simulink model "fullCarModel"  (R2024b)
settings: Solver=ode45  StartTime=0.0  StopTime=10.0  RelTol=1e-3  EnableMultiTasking=on
undefined symbols (not defined in the file or in its folder): sigbuilder_block
(part 1 of 2)
settings Model: Creator=Muhammad  LastModifiedBy=ryuu1
settings SolverCC: AlgebraicLoopSolver=TrustRegion
settings DataIOCC: LimitDataPoints=on  SaveFormat=Array  ReturnWorkspaceOutputs=off
settings OptimizationCC: LifeSpan=inf
settings DebuggingCC: UnderspecifiedInitializationDetection=Classic  MergeDetectMultiDrivingBlocksExec=none  SolverPrmCheckMsg=warning  UnconnectedInputMsg=warning  UnconnectedOutputMsg=warning  UnconnectedLineMsg=warning  StateNameClashWarn=warning  SFUnexpectedBacktrackingDiag=warning  SFNoUnconditionalDefaultTransitionDiag=warning  SFExecutionAtInitializationDiag=none  ArithmeticOperatorsInVariantConditions=warning
settings HardwareCC: ProdBitPerPointer=32  ProdBitPerSizeT=32  ProdBitPerPtrDiffT=32  ProdLargestAtomicFloat=None  ProdIntDivRoundTo=Undefined  ProdEndianess=Unspecified  ProdWordSize=32  ProdHWDeviceType=32-bit Generic
settings ModelReferenceCC: PropagateSignalLabelsOutOfModel=off
settings SFSimCC: SimUseLocalCustomCode=off  CustomCodeUndefinedFunction=UseInterfaceOnly
settings RTWCC: RTWUseLocalCustomCode=off  GPUComputeCapability=3.5
settings CodeAppCC: StateflowObjectComments=on
settings GRTTargetCC: TargetLangStandard=C89/C90 (ANSI)
settings ConfigComp: CovMetricSettings=dw  CovSaveCumulativeToWorkspaceVar=on  CovSaveSingleToWorkspaceVar=on  CovExternalEMLEnable=off

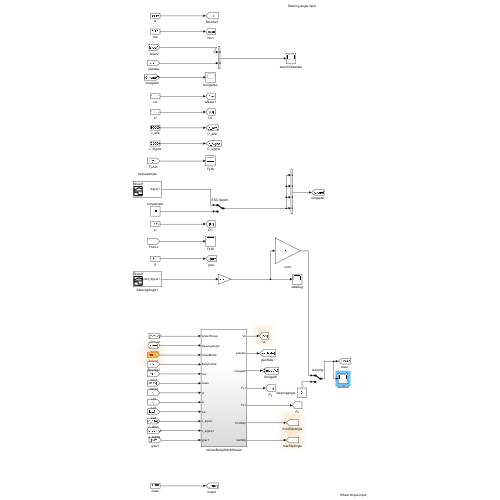
[thumbnail: Simulink's stored preview of the top-level diagram]
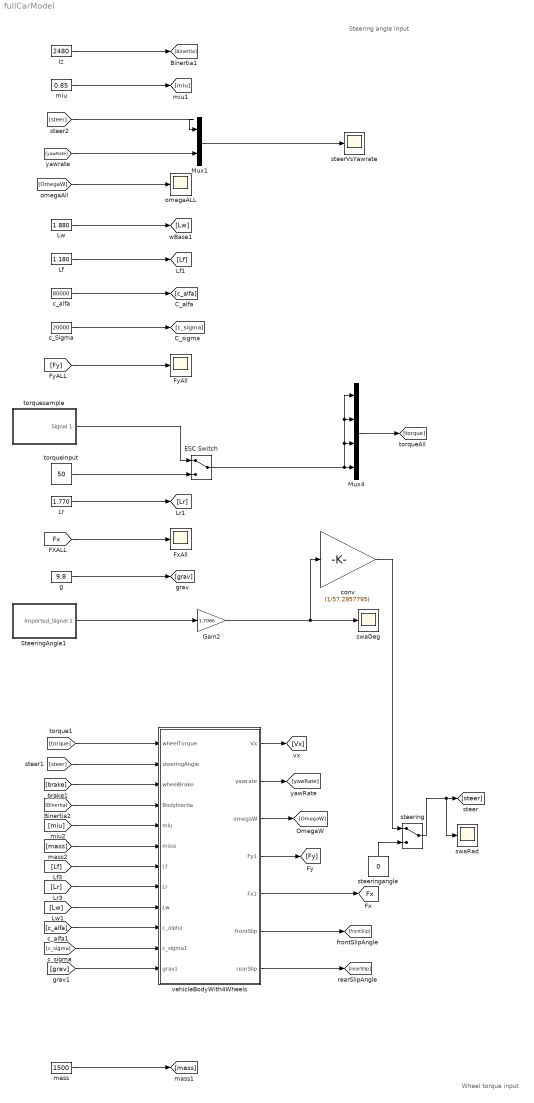
== system fullCarModel ==
  note: Wheel torque input
  note: Steering angle input
  ESC Switch : ManualSwitch
  FxAll : Scope
  FyAll : Scope
  Gain2 : Gain  Gain=1.7086
  Iz : Constant  Value=2480
  Lf : Constant  Value=1.180
  Lr : Constant  Value=1.770
  Lw : Constant  Value=1.880
  Mux1 : Mux  Inputs=2
      settings: DisplayOption=signals
  Mux4 : Mux
      settings: DisplayOption=signals
  SteeringAngle1 : Subsystem  Tag=STV Subsys  LoadFcn=sigbuilder_block('load');  StartFcn=sigbuilder_block('start');  StopFcn=sigbuilder_block('stop');  ClipboardFcn=sigbuilder_block('clipboard');  mask(Sigbuilder block){tuvar=[0:10]}
      mask help: Create and generate interchangeable groups of signals whose waveforms are piecewise linear.
      mask init:
      | if ~strcmp(get_param(bdroot(gcbh),'SimulationStatus'),'stopped') tuvar = sigbuilder_block('maskInit'); end
      settings: CopyFcn=sigbuilder_block('copy');  DeleteFcn=sigbuilder_block('delete');  ModelCloseFcn=sigbuilder_block('modelClose');  PreSaveFcn=sigbuilder_block('preSave');  PauseFcn=sigbuilder_block('pause')  ContinueFcn=sigbuilder_block('continue')  NameChangeFcn=sigbuilder_block('namechange');  OpenFcn=sigbuilder_block('open',[339.75 9 678.75 504 ]);  CloseFcn=sigbuilder_block('close');
      mask Display: plot(0, 0, 100, 100,[2, 2, 32, 32, 2], [68, 8, 8, 68, 68],[32, 2], [38, 38], [32, 19, 2],[53, 60, 44], [32, 17, 17, 2],[16, 16, 31, 31]);txt = getActiveGroup(gcbh);text(2, 100, txt,'verticalAlignment', 'top');
  c_Sigma : Constant  Value=20000
  c_alfa : Constant  Value=80000
  conv : Gain  Gain=(1/57.2957795)
  g : Constant  Value=9.8
  mass : Constant  Value=1500
  miu : Constant  Value=0.85
  omegaALL : Scope
  steerVsYawrate : Scope
  steering : ManualSwitch
  steeringangle : Constant  Value=0
  swaDeg : Scope
  swaRad : Scope
  torqueInput : Constant  Value=50
  "torquesample " : Subsystem  Tag=STV Subsys  LoadFcn=sigbuilder_block('load');  StartFcn=sigbuilder_block('start');  StopFcn=sigbuilder_block('stop');  ClipboardFcn=sigbuilder_block('clipboard');  mask(Sigbuilder block){tuvar=[0:10]}
      mask help: Create and generate interchangeable groups of signals whose waveforms are piecewise linear.
      mask init:
      | if ~strcmp(get_param(bdroot(gcbh),'SimulationStatus'),'stopped') tuvar = sigbuilder_block('maskInit'); end
      settings: CopyFcn=sigbuilder_block('copy');  DeleteFcn=sigbuilder_block('delete');  ModelCloseFcn=sigbuilder_block('modelClose');  PreSaveFcn=sigbuilder_block('preSave');  PauseFcn=sigbuilder_block('pause')  ContinueFcn=sigbuilder_block('continue')  NameChangeFcn=sigbuilder_block('namechange');  OpenFcn=sigbuilder_block('open',[6 28.5 1012.5 484.5 ]);  CloseFcn=sigbuilder_block('close');
      mask Display: plot(0, 0, 100, 100,[2, 2, 32, 32, 2], [68, 8, 8, 68, 68],[32, 2], [38, 38], [32, 19, 2],[53, 60, 44], [32, 17, 17, 2],[16, 16, 31, 31]);txt = getActiveGroup(gcbh);text(2, 100, txt,'verticalAlignment', 'top');
  vehicleBodyWith4Wheels : Subsystem
  tag scope: Fx=global
  wires:
  [steer] -> Mux1/1
  [Fy] -> FyAll/1
  Iz/1 -> [Binertia]
  miu/1 -> [miu]
  Lw/1 -> [Lw]
  Lf/1 -> [Lf]
  vehicleBodyWith4Wheels/5(Fx1) -> [Fx]
  vehicleBodyWith4Wheels/1(Vx) -> [Vx]
  [yawRate] -> Mux1/2
  ESC Switch/1 -> Mux4/2, Mux4/1, Mux4/3, Mux4/4
  [OmegaW] -> omegaALL/1
  Gain2/1 -> swaDeg/1, conv/1
  [c_sigma] -> vehicleBodyWith4Wheels/11(c_sigma1)
  c_alfa/1 -> [c_alfa]
  [mass] -> vehicleBodyWith4Wheels/6(mass)
  c_Sigma/1 -> [c_sigma]
  "torquesample "/1(Signal 1) -> ESC Switch/1
  steering/1 -> swaRad/1, [steer]
  [torque] -> vehicleBodyWith4Wheels/1(wheelTorque)
  torqueInput/1 -> ESC Switch/2
  [Lr] -> vehicleBodyWith4Wheels/8(Lr)
  Lr/1 -> [Lr]
  [Fx] -> FxAll/1
  [grav] -> vehicleBodyWith4Wheels/12(grav1)
  g/1 -> [grav]
  Mux4/1 -> [torque]
  Mux1/1 -> steerVsYawrate/1
  SteeringAngle1/1(Imported_Signal 1) -> Gain2/1
  conv/1 -> steering/1
  [steer] -> vehicleBodyWith4Wheels/2(steeringAngle)
  [brake] -> vehicleBodyWith4Wheels/3(wheelBrake)
  [Binertia] -> vehicleBodyWith4Wheels/4(BodyInertia)
  [miu] -> vehicleBodyWith4Wheels/5(miu)
  [Lf] -> vehicleBodyWith4Wheels/7(Lf)
  [Lw] -> vehicleBodyWith4Wheels/9(Lw)
  [c_alfa] -> vehicleBodyWith4Wheels/10(c_alpha)
  mass/1 -> [mass]
  vehicleBodyWith4Wheels/6(frontSlip) -> [frontSlip]
  vehicleBodyWith4Wheels/2(yawrate) -> [yawRate]
  vehicleBodyWith4Wheels/7(rearSlip) -> [rearSlip]
  vehicleBodyWith4Wheels/3(omegaW) -> [OmegaW]
  vehicleBodyWith4Wheels/4(Fy1) -> [Fy]
  steeringangle/1 -> steering/2

== system fullCarModel/SteeringAngle1 ==
  Demux : Demux  Tag=STV Demux  Outputs=1
      settings: DisplayOption=none
  FromWs : FromWorkspace  Tag=STV FromWs  VariableName=tuvar
      SigBuilderData=|
      | common.afterFinalStr = 'Extrapolate'
      | common.sampleTime = 0
      | dataSet.timeRange = [0 22.075001]
      | dataSet.name = 'Sheet1'
      | sbobj.Name = 'Signal Builder'
      | sbobj.Groups.Name = 'Sheet1'
      | sbobj.Groups.Signals.Name = 'Imported_Signal 1'
      | sbobj.Groups.Signals.XData = [0 8.825 8.85 8.875 8.900001 8.925 8.95 8.975 9 9.025001 9.05 9.075 9.1 9.125 9.150001 9.175 9.2 9.225 9.25 9.275001 9.3 9.325 9.35 9.375 9.400001 9.425 9.45 9.475 9.5 9.525001 9.55 9.575 9.6 9.625 9.650001 9.675 9.7 9.725 9.75 9.775001 9.8 9.825 9.85 9.875 9.900001 9.925 9.95 9.975 10 10.025001 10.05 10.075 10.1 10.125 10.150001 10.175 10.2 10.225 10.25 10.275001 10.3 10.325 10.35 10.375 10.400001 10.425 10.45 10.475 10.5 10.525001 10.55 10.575 10.6 10.625 10.650001 10.675 10.7 10.725 10.75 10.775001 10.8 10.825 10.85 10.875 10.900001 10.925 10.95 10.975 11 11.025001 11.05 11.075 11.1 11.125 11.150001 11.175 11.2 11.225 11.25 11.275001 11.3 11.325 11.35 11.375 11.400001 11.425 11.45 11.475 11.5 11.525001 11.55 11.575 11.6 11.625 11.650001 11.675 11.7 11.725 11.75 11.775001 11.8 11.825 11.85 11.875 11.900001 11.925 11.95 11.975 12 12.025001 12.05 12.075 12.1 12.125 12.150001 12.175 12.2 12.225 12.25 12.275001 12.3 12.325 12.35 12.375 12.400001 12.425 12.45 12.475 12.5 12.525001 12.55 12.575 12.6 12.625 12.650001 12.675 12.7 12.725 12.75 12.775001 12.8 12.825 12.85 12.875 12.900001 12.925 12.95 12.975 13 13.025001 13.05 13.075 13.1 13.125 13.150001 13.175 13.2 13.225 13.25 13.275001 13.3 13.325 13.35 13.375 13.400001 13.425 13.45 13.475 13.5 13.525001 13.55 13.575 13.6 13.625 13.650001 13.675 13.7 13.725 13.75 13.775001 13.8 13.825 13.85 13.875 13.900001 13.925 13.95 13.975 21.85 21.875 21.9 21.925001 21.950001 21.975 22 22.025 22.050001 22.075001]
      | sbobj.Groups.Signals.YData = [0 0.062882 0.050573 0.039906 2.188617 9.974806 17.646795 25.09313 32.23859 39.002769 45.307468 51.033176 56.152084 60.606716 64.344048 67.25927 69.377258 70.674423 71.133003 70.682831 69.396751 67.289543 64.38208 60.65221 56.206863 51.096375 45.376297 39.076691 32.318226 25.177221 17.73332 10.063081 2.277949 -5.534312 -13.285121 -20.865993 -28.195927 -35.192413 -41.774796 -47.823311 -53.302822 -58.151779 -62.312809 -65.677658 -68.263748 -70.042198 -70.98983 -71.000824 -71.007645 -71.014473 -71.021294 -71.028114 -71.034943 -71.041763 -71.048584 -71.055412 -71.062233 -71.069054 -71.075882 -71.082703 -71.089531 -71.096352 -71.103172 -71.110001 -71.116821 -71.123642 -71.13047 -71.030533 -70.230949 -68.600365 -66.154236 -62.863037 -58.829971 -54.100742 -48.726452 -42.72982 -36.230957 -29.303261 -22.023787 -14.463158 -6.735525 0 0 0 0 0 0 0 0 0 0 0 0 0 0 0 0 0 0 0 0 0 0 0 0 0 0 0 0 0 0 0 0 0 0 0 0 0 0 0 0 0 0 0 0 0 0 0 0 0 0 0 0 0 0 0 0 0 0 0 0 0 0 0 0 0 0 0 0 0 0 0.053113 -0.021248 -0.028092 -0.032833 -0.036965 -0.040874 -0.044865 -0.049055 -0.053398 -0.05781 -0.062213 -0.066522 -0.070706 -0.07473 -0.078582 -0.082254 -0.085717 -0.089006 -0.092088 -0.095001 -0.097757 -0.100312 -0.105833 -0.099933 -0.080947 -0.064335 -0.050307 -0.038064 -0.027431 -0.017977 -0.009421 -0.001665 0.005429 0.012031 0.018383 0.024606 0.030729 0.036764 0.042774 0.048745 0.05465 0.060456 0.066071 0.071523 0.076801 0.081817 0.086576 0.091128 0.09541 0.099418 0.105225 0.105563 0.089248 0.072885 0.059331 0.047486 0.037205 0 0 0 0 0 0 0 0 0 0]
      | sbobj.Groups.TimeRange = [0 22.075001]
  Imported_Signal 1 : Outport  Tag=STV Outport
  wires:
  FromWs/1 -> Demux/1
  Demux/1 -> Imported_Signal 1/1

== system fullCarModel/torquesample  ==
  Demux : Demux  Tag=STV Demux  Outputs=1
      settings: DisplayOption=none
  FromWs : FromWorkspace  Tag=STV FromWs  VariableName=tuvar
      SigBuilderData=|
      | common.afterFinalStr = 'Extrapolate'
      | common.sampleTime = 0
      | dataSet.timeRange = [0 22.075001]
      | dataSet.name = 'Sheet1'
      | sbobj.Name = 'Signal Builder'
      | sbobj.Groups.Name = 'Sheet1'
      | sbobj.Groups.Signals.Name = 'Signal 1'
      | sbobj.Groups.Signals.XData = [0 0.5 1 1 22.075001]
      | sbobj.Groups.Signals.YData = [0 50 50 0 0]
      | sbobj.Groups.TimeRange = [0 22.075001]
  Signal 1 : Outport  Tag=STV Outport
  wires:
  FromWs/1 -> Demux/1
  Demux/1 -> Signal 1/1

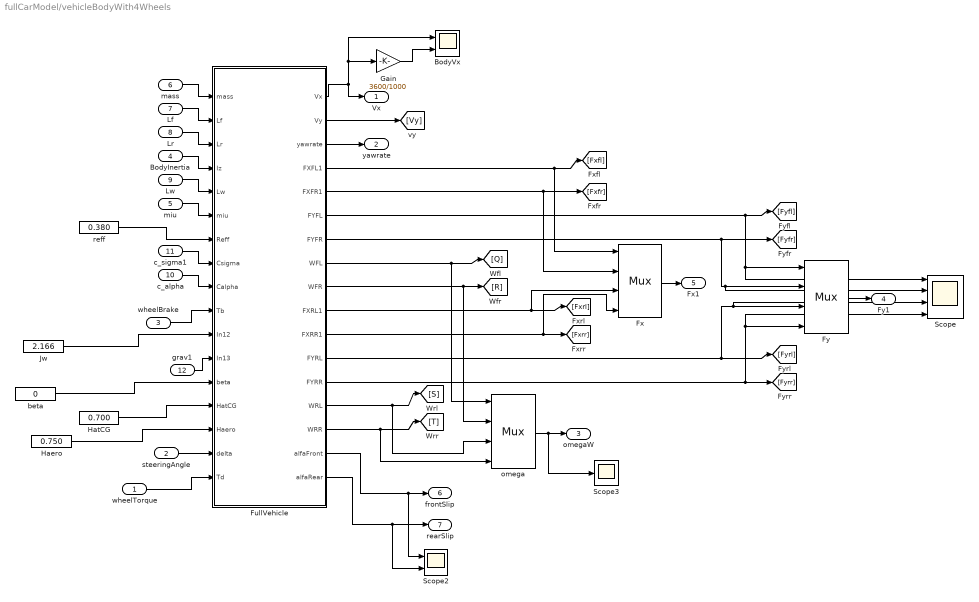
== system fullCarModel/vehicleBodyWith4Wheels ==
  wheelTorque : Inport
  steeringAngle : Inport  Port=2
  wheelBrake : Inport  Port=3
  BodyInertia : Inport  Port=4
  miu : Inport  Port=5
  mass : Inport  Port=6
  Lf : Inport  Port=7
  Lr : Inport  Port=8
  Lw : Inport  Port=9
  c_alpha : Inport  Port=10
  c_sigma1 : Inport  Port=11
  grav1 : Inport  Port=12
  BodyVx : Scope  NumInputPorts=2
  FullVehicle : Subsystem
  Fx : Mux
  Fy : Mux
  Gain : Gain  Gain=3600/1000
  Haero : Constant  Value=0.750
  HatCG : Constant  Value=0.700
  Jw : Constant  Value=2.166
  Scope : Scope  NumInputPorts=4
  Scope2 : Scope  NumInputPorts=2
  Scope3 : Scope
  beta : Constant  Value=0
  omega : Mux
  reff : Constant  Value=0.380
  Vx : Outport
  yawrate : Outport  Port=2
  omegaW : Outport  Port=3
  Fy1 : Outport  Port=4
  Fx1 : Outport  Port=5
  frontSlip : Outport  Port=6
  rearSlip : Outport  Port=7
  wires:
  Lw/1 -> FullVehicle/5(Lw)
  Jw/1 -> FullVehicle/11(In12)
  reff/1 -> FullVehicle/7(Reff)
  beta/1 -> FullVehicle/13(beta)
  HatCG/1 -> FullVehicle/14(HatCG)
  Haero/1 -> FullVehicle/15(Haero)
  FullVehicle/1(Vx) -> BodyVx/1, Gain/1, Vx/1
  FullVehicle/2(Vy) -> [Vy]
  FullVehicle/3(yawrate) -> yawrate/1
  FullVehicle/4(FXFL1) -> [Fxfl], Fx/1
  FullVehicle/5(FXFR1) -> [Fxfr], Fx/2
  FullVehicle/6(FYFL) -> [Fyfl], Fy/1, Scope/1
  FullVehicle/7(FYFR) -> [Fyfr], Fy/2, Scope/2
  FullVehicle/8(WFL) -> [Q], omega/1
  FullVehicle/9(WFR) -> [R], omega/2
  FullVehicle/10(FXRL1) -> [Fxrl], Fx/3
  FullVehicle/11(FXRR1) -> [Fxrr], Fx/4
  FullVehicle/12(FYRL) -> [Fyrl], Fy/3, Scope/3
  FullVehicle/13(FYRR) -> [Fyrr], Fy/4, Scope/4
  FullVehicle/14(WRL) -> [S], omega/3
  FullVehicle/15(WRR) -> [T], omega/4
  FullVehicle/16(alfaFront) -> frontSlip/1, Scope2/1
  FullVehicle/17(alfaRear) -> rearSlip/1, Scope2/2
  steeringAngle/1 -> FullVehicle/16(delta)
  wheelTorque/1 -> FullVehicle/17(Td)
  wheelBrake/1 -> FullVehicle/10(Tb)
  omega/1 -> Scope3/1, omegaW/1
  Fy/1 -> Fy1/1
  Fx/1 -> Fx1/1
  BodyInertia/1 -> FullVehicle/4(Iz)
  miu/1 -> FullVehicle/6(miu)
  mass/1 -> FullVehicle/1(mass)
  Lf/1 -> FullVehicle/2(Lf)
  Lr/1 -> FullVehicle/3(Lr)
  c_alpha/1 -> FullVehicle/9(Calpha)
  c_sigma1/1 -> FullVehicle/8(Csigma)
  grav1/1 -> FullVehicle/12(In13)
  Gain/1 -> BodyVx/2

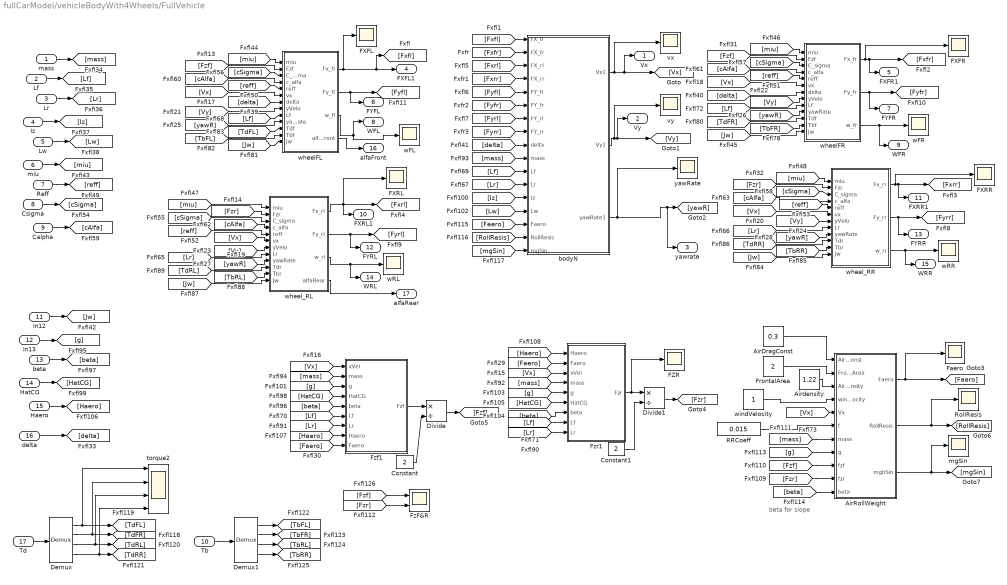
== system fullCarModel/vehicleBodyWith4Wheels/FullVehicle ==
  note: beta for slope
  mass : Inport
  Lf : Inport  Port=2
  Lr : Inport  Port=3
  Iz : Inport  Port=4
  Lw : Inport  Port=5
  miu : Inport  Port=6
  Reff : Inport  Port=7
  Csigma : Inport  Port=8
  Calpha : Inport  Port=9
  Tb : Inport  Port=10
  In12 : Inport  Port=11
  In13 : Inport  Port=12
  beta : Inport  Port=13
  HatCG : Inport  Port=14
  Haero : Inport  Port=15
  delta : Inport  Port=16
  Td : Inport  Port=17
  AirDragConst : Constant  Value=0.3
  AirRollWeight : Subsystem
  Airdensity : Constant  Value=1.22
  Constant : Constant  Value=2
  Constant1 : Constant  Value=2
  Demux : Demux
      settings: DisplayOption=none
  Demux1 : Demux
      settings: DisplayOption=none
  Divide : Product  Inputs=*/
  Divide1 : Product  Inputs=*/
  FXFL : Scope
  FXFR : Scope
  FXRL : Scope
  FXRR : Scope
  FZR : Scope
  Faero : Scope
  FrontalArea : Constant  Value=2
  FzF&R : Scope  NumInputPorts=2
  Fzf1 : Subsystem
  Fzr1 : Subsystem
  RRCoeff : Constant  Value=0.015
  RollResis : Scope
  bodyN : Subsystem
  mgSin : Scope
  torque2 : Scope  NumInputPorts=4
  vx : Scope
  vy : Scope
  wFL : Scope
  wFR : Scope
  wRL : Scope
  wRR : Scope
  wheelFL : Subsystem
  wheelFR : Subsystem
  wheel_RL : Subsystem
  wheel_RR : Subsystem
  windVelocity : Constant
  yawRate : Scope
  Vx : Outport
  Vy : Outport  Port=2
  yawrate : Outport  Port=3
  FXFL1 : Outport  Port=4
  FXFR1 : Outport  Port=5
  FYFL : Outport  Port=6
  FYFR : Outport  Port=7
  WFL : Outport  Port=8
  WFR : Outport  Port=9
  FXRL1 : Outport  Port=10
  FXRR1 : Outport  Port=11
  FYRL : Outport  Port=12
  FYRR : Outport  Port=13
  WRL : Outport  Port=14
  WRR : Outport  Port=15
  alfaFront : Outport  Port=16
  alfaRear : Outport  Port=17
  wires:
  wheelFL/1(Fx_fl) -> FXFL/1, [Fxfl], FXFL1/1
  wheel_RL/1(Fx_rl) -> [Fxrl], FXRL1/1, FXRL/1
  wheel_RR/1(Fx_rr) -> FXRR/1, [Fxrr], FXRR1/1
  [Fxrl] -> bodyN/3(FX_rl)
  [Fxrr] -> bodyN/4(FX_rr)
  [Fxfr] -> bodyN/2(FX_fr)
  [Fxfl] -> bodyN/1(FX_fl)
  [Fyfl] -> bodyN/5(FY_fl)
  [Fyfr] -> bodyN/6(FY_fr)
  [Fyrl] -> bodyN/7(FY_rl)
  [Fyrr] -> bodyN/8(FY_rr)
  [delta] -> bodyN/9(delta)
  [mass] -> bodyN/10(mass)
  [Lr] -> bodyN/12(Lr)
  [Lw] -> bodyN/14(Lw)
  wheelFL/2(Fy_fl) -> [Fyfl], FYFL/1
  wheel_RL/2(Fy_rl) -> [Fyrl], FYRL/1
  wheel_RR/2(Fy_rr) -> [Fyrr], FYRR/1
  bodyN/1(Vx1) -> vx/1, [Vx], Vx/1
  bodyN/2(Vy1) -> vy/1, [Vy], Vy/1
  [Vx] -> wheelFL/6(vx)
  [Vy] -> wheelFL/8(yVelo)
  [Vx] -> wheel_RL/6(vx)
  [Vy] -> wheel_RL/7(yVelo)
  [Vx] -> wheel_RR/6(vx)
  [Vy] -> wheel_RR/7(yVelo)
  [Vx] -> Fzr1/3(xVel)
  [Vx] -> Fzf1/1(xVel)
  [yawR] -> wheelFL/10(yawRate)
  [yawR] -> wheel_RL/9(yawRate)
  [yawR] -> wheel_RR/9(yawRate)
  [Faero] -> Fzf1/9(Faero)
  [Faero] -> Fzr1/2(Faero)
  Fzr1/1(Fzr) -> Divide1/1, FZR/1
  Fzf1/1(Fzf) -> Divide/1
  [Fzf] -> wheelFL/2(Fzf)
  [Fzr] -> wheel_RL/2(Fzr)
  [Fzr] -> wheel_RR/2(Fzr)
  [miu] -> wheelFL/1(miu)
  [miu] -> wheel_RL/1(miu)
  [miu] -> wheel_RR/1(miu)
  [reff] -> wheelFL/5(reff)
  [reff] -> wheel_RL/5(reff)
  [cSigma] -> wheelFL/3(C_sigma)
  [cSigma] -> wheel_RR/3(C_sigma)
  [cSigma] -> wheel_RL/3(C_sigma)
  [cAlfa] -> wheelFL/4(c_alfa)
  [cAlfa] -> wheel_RL/4(c_alfa)
  [cAlfa] -> wheel_RR/4(c_alfa)
  [delta] -> wheelFL/7(delta)
  [Lf] -> Fzr1/8(Lf)
  [Lf] -> bodyN/11(Lf)
  [Lr] -> wheel_RL/8(Lr)
  [reff] -> wheel_RR/5(reff)
  [Lr] -> wheel_RR/8(Lr)
  [Lf] -> wheelFL/9(Lf)
  [TdRR] -> wheel_RR/10(Tdr)
  [TbRR] -> wheel_RR/11(Tbr)
  [Jw] -> wheel_RR/12(Jw)
  [TdRL] -> wheel_RL/10(Tdr)
  [TbRL] -> wheel_RL/11(Tbr)
  [Jw] -> wheel_RL/12(Jw)
  [TdFL] -> wheelFL/11(Tdf)
  [TbFL] -> wheelFL/12(Tbf)
  [Jw] -> wheelFL/13(Jw)
  [Lr] -> Fzr1/9(Lr)
  [Lr] -> Fzf1/7(Lr)
  [Lf] -> Fzf1/6(Lf)
  [mass] -> Fzr1/4(mass)
  [mass] -> Fzf1/2(mass)
  [Iz] -> bodyN/13(Iz)
  [g] -> Fzr1/5(g)
  [HatCG] -> Fzr1/6(HatCG)
  [beta] -> Fzr1/7(beta)
  [g] -> Fzf1/3(g)
  [HatCG] -> Fzf1/4(HatCG)
  [beta] -> Fzf1/5(beta)
  [Haero] -> Fzf1/8(Haero)
  [Haero] -> Fzr1/1(Haero)
  wheelFL/3(w_fl) -> wFL/1, WFL/1
  wheel_RR/3(w_rr) -> wRR/1, WRR/1
  wheel_RL/3(w_rl) -> wRL/1, WRL/1
  wheelFR/1(Fx_fr) -> FXFR/1, [Fxfr], FXFR1/1
  wheelFR/2(Fy_fr) -> [Fyfr], FYFR/1
  [Vx] -> wheelFR/6(vx)
  [Vy] -> wheelFR/8(yVelo)
  [yawR] -> wheelFR/10(yawRate)
  [Fzf] -> wheelFR/2(Fzf)
  [miu] -> wheelFR/1(miu)
  [reff] -> wheelFR/5(reff)
  [cSigma] -> wheelFR/3(C_sigma)
  [cAlfa] -> wheelFR/4(c_alfa)
  [delta] -> wheelFR/7(delta)
  [Lf] -> wheelFR/9(Lf)
  [TdFR] -> wheelFR/11(Tdf)
  [TbFR] -> wheelFR/12(Tbf)
  [Jw] -> wheelFR/13(Jw)
  wheelFR/3(w_fr) -> wFR/1, WFR/1
  Divide/1 -> [Fzf]
  Constant/1 -> Divide/2
  Divide1/1 -> [Fzr]
  Constant1/1 -> Divide1/2
  [Faero] -> bodyN/15(Faero)
  [RollResis] -> bodyN/16(RollResis)
  [mgSin] -> bodyN/17(mgSin)
  mass/1 -> [mass]
  Lf/1 -> [Lf]
  Lr/1 -> [Lr]
  Iz/1 -> [Iz]
  Lw/1 -> [Lw]
  miu/1 -> [miu]
  Reff/1 -> [reff]
  Csigma/1 -> [cSigma]
  Calpha/1 -> [cAlfa]
  In12/1 -> [Jw]
  In13/1 -> [g]
  beta/1 -> [beta]
  HatCG/1 -> [HatCG]
  Haero/1 -> [Haero]
  delta/1 -> [delta]
  wheelFL/4(alfaFront) -> alfaFront/1
  wheel_RL/4(alfaRear) -> alfaRear/1
  Demux/1 -> [TdFL], torque2/1
  Demux/2 -> [TdFR], torque2/2
  Demux/3 -> [TdRL], torque2/3
  Demux/4 -> [TdRR], torque2/4
  Td/1 -> Demux/1
  Demux1/1 -> [TbFL]
  Demux1/2 -> [TbFR]
  Demux1/3 -> [TbRL]
  Demux1/4 -> [TbRR]
  Tb/1 -> Demux1/1
  [Fzr] -> FzF&R/2
  [Fzf] -> FzF&R/1
  bodyN/3(yawRate1) -> yawRate/1, [yawR], yawrate/1
  AirDragConst/1 -> AirRollWeight/1(AirDragConst)
  FrontalArea/1 -> AirRollWeight/2(FrontalArea)
  windVelocity/1 -> AirRollWeight/4(windVelocity)
  Airdensity/1 -> AirRollWeight/3(Airdensity)
  [Vx] -> AirRollWeight/5(Vx)
  AirRollWeight/1(Faero) -> [Faero], Faero/1
  [mass] -> AirRollWeight/7(mass)
  [Fzf] -> AirRollWeight/9(fzf)
  [Fzr] -> AirRollWeight/10(fzr)
  [g] -> AirRollWeight/8(g)
  [beta] -> AirRollWeight/11(beta)
  RRCoeff/1 -> AirRollWeight/6(f)
  AirRollWeight/2(RollResis) -> [RollResis], RollResis/1
  AirRollWeight/3(mghSin) -> [mgSin], mgSin/1

== system fullCarModel/vehicleBodyWith4Wheels/FullVehicle/AirRollWeight ==
  AirDragConst : Inport
  FrontalArea : Inport  Port=2
  Airdensity : Inport  Port=3
  windVelocity : Inport  Port=4
  Vx : Inport  Port=5
  f : Inport  Port=6
  mass : Inport  Port=7
  g : Inport  Port=8
  fzf : Inport  Port=9
  fzr : Inport  Port=10
  beta : Inport  Port=11
  Add : Sum
  Constant : Constant  Value=2
  Faero1 : Subsystem
  Product : Product  Inputs=3  RndMeth=Zero
  Product1 : Product  RndMeth=Zero
  Product2 : Product  RndMeth=Zero
  Trigonometric Function : Trigonometry
  Faero : Outport
  RollResis : Outport  Port=2
  mghSin : Outport  Port=3
  wires:
  AirDragConst/1 -> Faero1/1(AirDragConst1)
  FrontalArea/1 -> Faero1/2(FrontalArea1)
  windVelocity/1 -> Faero1/4(windVelocity)
  Airdensity/1 -> Faero1/3(Airdensity)
  Vx/1 -> Faero1/5(Vx)
  Faero1/1(Faero) -> Faero/1
  fzr/1 -> Add/1
  fzf/1 -> Add/2
  Add/1 -> Product/1
  f/1 -> Product/2
  Product/1 -> RollResis/1
  mass/1 -> Product1/1
  g/1 -> Product1/2
  beta/1 -> Trigonometric Function/1
  Product1/1 -> Product2/1
  Trigonometric Function/1 -> Product2/2
  Product2/1 -> mghSin/1
  Constant/1 -> Product/3

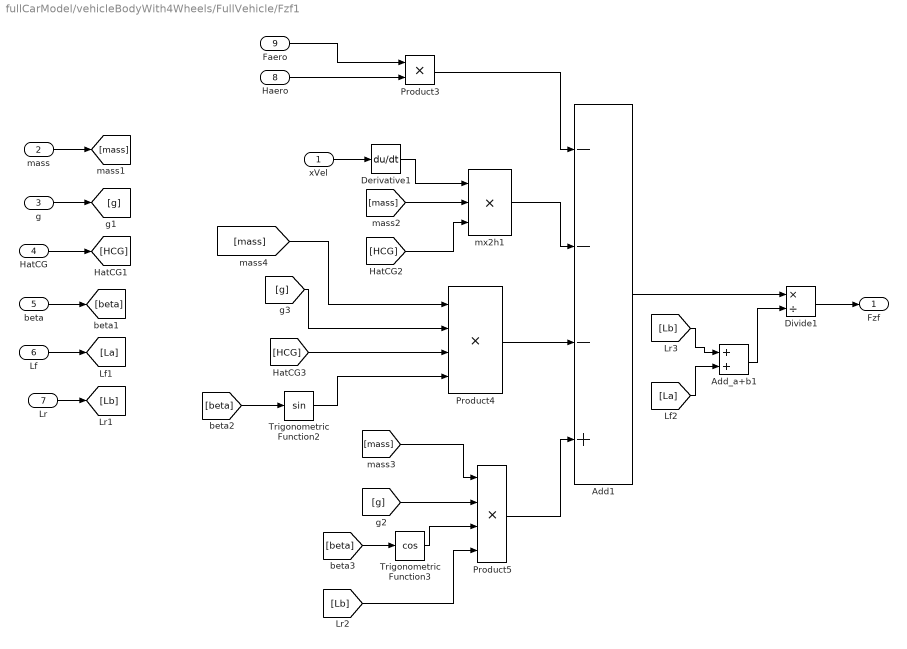
== system fullCarModel/vehicleBodyWith4Wheels/FullVehicle/Fzf1 ==
  xVel : Inport
  mass : Inport  Port=2
  g : Inport  Port=3
  HatCG : Inport  Port=4
  beta : Inport  Port=5
  Lf : Inport  Port=6
  Lr : Inport  Port=7
  Haero : Inport  Port=8
  Faero : Inport  Port=9
  Add1 : Sum  Inputs=---+
  Add_a+b1 : Sum
  Derivative1 : Derivative
  Divide1 : Product  Inputs=*/
  Product3 : Product  RndMeth=Zero
  Product4 : Product  Inputs=4  RndMeth=Zero
  Product5 : Product  Inputs=4  RndMeth=Zero
  Trigonometric Function2 : Trigonometry
  Trigonometric Function3 : Trigonometry  Operator=cos
  mx2h1 : Product  Inputs=3  RndMeth=Zero
  Fzf : Outport
  wires:
  Derivative1/1 -> mx2h1/1
  [HCG] -> mx2h1/3
  [beta] -> Trigonometric Function2/1
  [beta] -> Trigonometric Function3/1
  [HCG] -> Product4/3
  Trigonometric Function2/1 -> Product4/4
  [mass] -> Product5/1
  Trigonometric Function3/1 -> Product5/3
  [Lb] -> Product5/4
  [Lb] -> Add_a+b1/1
  [La] -> Add_a+b1/2
  Product3/1 -> Add1/1
  mx2h1/1 -> Add1/2
  Product4/1 -> Add1/3
  Product5/1 -> Add1/4
  Add1/1 -> Divide1/1
  Add_a+b1/1 -> Divide1/2
  Divide1/1 -> Fzf/1
  xVel/1 -> Derivative1/1
  [mass] -> Product4/1
  [g] -> Product4/2
  [mass] -> mx2h1/2
  [g] -> Product5/2
  mass/1 -> [mass]
  g/1 -> [g]
  HatCG/1 -> [HCG]
  beta/1 -> [beta]
  Lf/1 -> [La]
  Lr/1 -> [Lb]
  Faero/1 -> Product3/1
  Haero/1 -> Product3/2

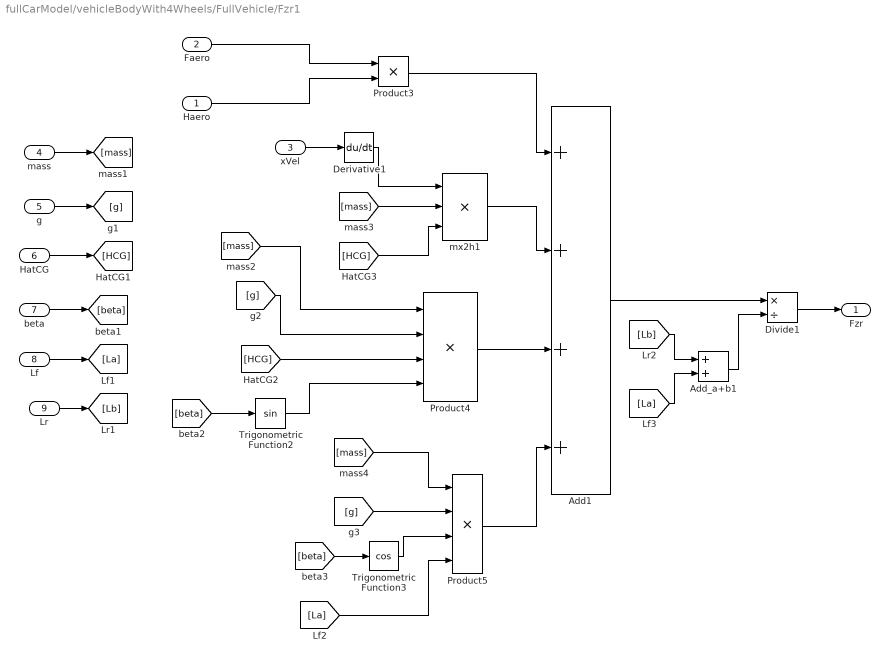
== system fullCarModel/vehicleBodyWith4Wheels/FullVehicle/Fzr1 ==
  Haero : Inport
  Faero : Inport  Port=2
  xVel : Inport  Port=3
  mass : Inport  Port=4
  g : Inport  Port=5
  HatCG : Inport  Port=6
  beta : Inport  Port=7
  Lf : Inport  Port=8
  Lr : Inport  Port=9
  Add1 : Sum  Inputs=++++
  Add_a+b1 : Sum
  Derivative1 : Derivative
  Divide1 : Product  Inputs=*/
  Product3 : Product  RndMeth=Zero
  Product4 : Product  Inputs=4  RndMeth=Zero
  Product5 : Product  Inputs=4  RndMeth=Zero
  Trigonometric Function2 : Trigonometry
  Trigonometric Function3 : Trigonometry  Operator=cos
  mx2h1 : Product  Inputs=3  RndMeth=Zero
  Fzr : Outport
  wires:
  Lr/1 -> [Lb]
  Lf/1 -> [La]
  beta/1 -> [beta]
  HatCG/1 -> [HCG]
  [g] -> Product5/2
  [mass] -> mx2h1/2
  [g] -> Product4/2
  g/1 -> [g]
  [mass] -> Product4/1
  mass/1 -> [mass]
  xVel/1 -> Derivative1/1
  Divide1/1 -> Fzr/1
  Add_a+b1/1 -> Divide1/2
  Add1/1 -> Divide1/1
  Product5/1 -> Add1/4
  Product4/1 -> Add1/3
  mx2h1/1 -> Add1/2
  Product3/1 -> Add1/1
  [La] -> Add_a+b1/2
  [Lb] -> Add_a+b1/1
  [La] -> Product5/4
  Trigonometric Function3/1 -> Product5/3
  [mass] -> Product5/1
  Trigonometric Function2/1 -> Product4/4
  [HCG] -> Product4/3
  [beta] -> Trigonometric Function3/1
  [beta] -> Trigonometric Function2/1
  [HCG] -> mx2h1/3
  Derivative1/1 -> mx2h1/1
  Haero/1 -> Product3/2
  Faero/1 -> Product3/1

== system fullCarModel/vehicleBodyWith4Wheels/FullVehicle/bodyN ==
  FX_fl : Inport
  FX_fr : Inport  Port=2
  FX_rl : Inport  Port=3
  FX_rr : Inport  Port=4
  FY_fl : Inport  Port=5
  FY_fr : Inport  Port=6
  FY_rl : Inport  Port=7
  FY_rr : Inport  Port=8
  delta : Inport  Port=9
  mass : Inport  Port=10
  Lf : Inport  Port=11
  Lr : Inport  Port=12
  Iz : Inport  Port=13
  Lw : Inport  Port=14
  Faero : Inport  Port=15
  RollResis : Inport  Port=16
  mgSin : Inport  Port=17
  Vx : Subsystem
  Vy : Subsystem
  yawRate : Subsystem
  Vx1 : Outport
  Vy1 : Outport  Port=2
  yawRate1 : Outport  Port=3
  wires:
  FX_fl/1 -> Vx/1(Fx_FL), Vy/1(Fx_FL), yawRate/1(Fx_FL)
  FX_fr/1 -> Vx/2(Fx_FR), Vy/2(Fx_FR), yawRate/2(Fx_FR)
  FX_rl/1 -> Vx/3(Fx_RL), yawRate/10(Fx_RL)
  FX_rr/1 -> Vx/4(Fx_RR), yawRate/11(Fx_RR)
  FY_fl/1 -> Vx/5(Fy_FL), Vy/5(Fy_FL), yawRate/5(Fy_FL)
  FY_fr/1 -> Vx/6(Fy_FR), Vy/6(Fy_FR), yawRate/6(Fy_FR)
  mass/1 -> Vx/7(mass), Vy/7(mass)
  delta/1 -> Vy/8(delta), yawRate/7(delta), Vx/8(delta)
  Vy/1(yVel) -> Vx/9(yVel), Vy1/1
  yawRate/1(yaw1) -> Vx/10(yaw1), Vy/10(yaw), yawRate1/1
  FY_rl/1 -> Vy/3(Fy_RL), yawRate/3(Fy_RL)
  FY_rr/1 -> Vy/4(Fy_RR), yawRate/4(Fy_RR)
  Lr/1 -> yawRate/9(Lr)
  Lf/1 -> yawRate/8(Lf)
  Vx/1(xVel) -> Vx1/1, Vy/9(xVel)
  Iz/1 -> yawRate/12(Iz)
  Lw/1 -> yawRate/13(Lw)
  Faero/1 -> Vx/11(Faero)
  RollResis/1 -> Vx/12(RollResis)
  mgSin/1 -> Vx/13(mgSin)

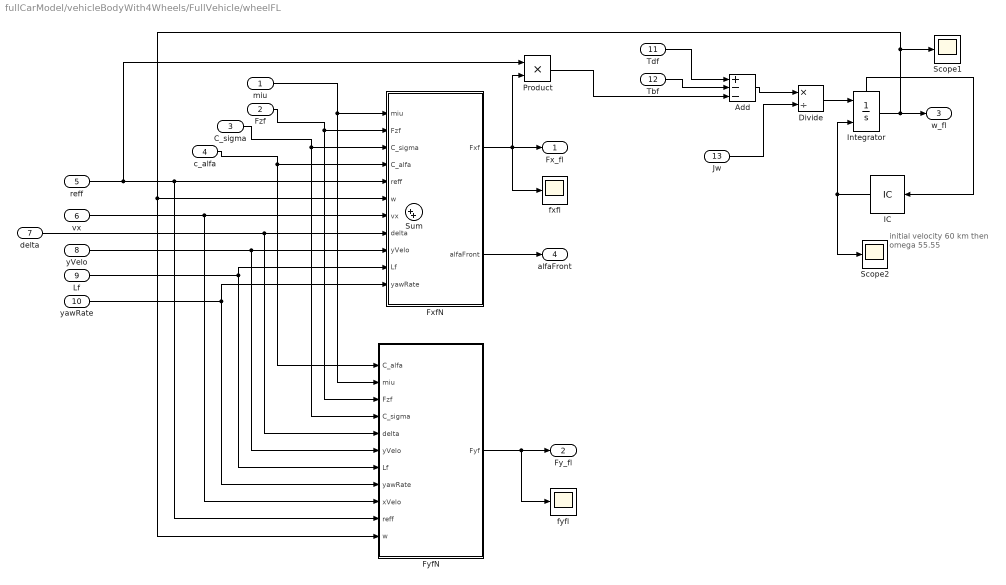
== system fullCarModel/vehicleBodyWith4Wheels/FullVehicle/wheelFL ==
  note: initial velocity 60 km then
      |  omega 55.55
  miu : Inport
  Fzf : Inport  Port=2
  C_sigma : Inport  Port=3
  c_alfa : Inport  Port=4
  reff : Inport  Port=5
  vx : Inport  Port=6
  delta : Inport  Port=7
  yVelo : Inport  Port=8
  Lf : Inport  Port=9
  yawRate : Inport  Port=10
  Tdf : Inport  Port=11
  Tbf : Inport  Port=12
  Jw : Inport  Port=13
  Add : Sum  Inputs=+--
  Divide : Product  Inputs=*/
  FxfN : Subsystem
  FyfN : Subsystem
  IC : InitialCondition  Value=55.55
  Integrator : Integrator  InitialConditionSource=external  ShowStatePort=on
  Product : Product  RndMeth=Zero
  Scope1 : Scope
  Scope2 : Scope
  Sum : Sum  Inputs=|++
  fxfl : Scope
  fyfl : Scope
  Fx_fl : Outport
  Fy_fl : Outport  Port=2
  w_fl : Outport  Port=3
  alfaFront : Outport  Port=4
  wires:
  miu/1 -> FxfN/1(miu), FyfN/2(miu)
  Fzf/1 -> FxfN/2(Fzf), FyfN/3(Fzf)
  C_sigma/1 -> FxfN/3(C_sigma), FyfN/4(C_sigma)
  c_alfa/1 -> FxfN/4(C_alfa), FyfN/1(C_alfa)
  reff/1 -> Product/1, FxfN/5(reff), FyfN/10(reff)
  vx/1 -> FxfN/7(vx), FyfN/9(xVelo)
  delta/1 -> FyfN/5(delta), FxfN/8(delta)
  yVelo/1 -> FyfN/6(yVelo), FxfN/9(yVelo)
  Lf/1 -> FxfN/10(Lf), FyfN/7(Lf)
  yawRate/1 -> FxfN/11(yawRate), FyfN/8(yawRate)
  FxfN/1(Fxf) -> Product/2, Fx_fl/1, fxfl/1
  FyfN/1(Fyf) -> fyfl/1, Fy_fl/1
  Tdf/1 -> Add/1
  Tbf/1 -> Add/2
  Product/1 -> Add/3
  Jw/1 -> Divide/2
  Add/1 -> Divide/1
  Divide/1 -> Integrator/1
  Integrator/1 -> Scope1/1, FxfN/6(w), FyfN/11(w), w_fl/1
  FxfN/2(alfaFront) -> alfaFront/1
  IC/1 -> Scope2/1, Integrator/2
  Integrator/State -> IC/1

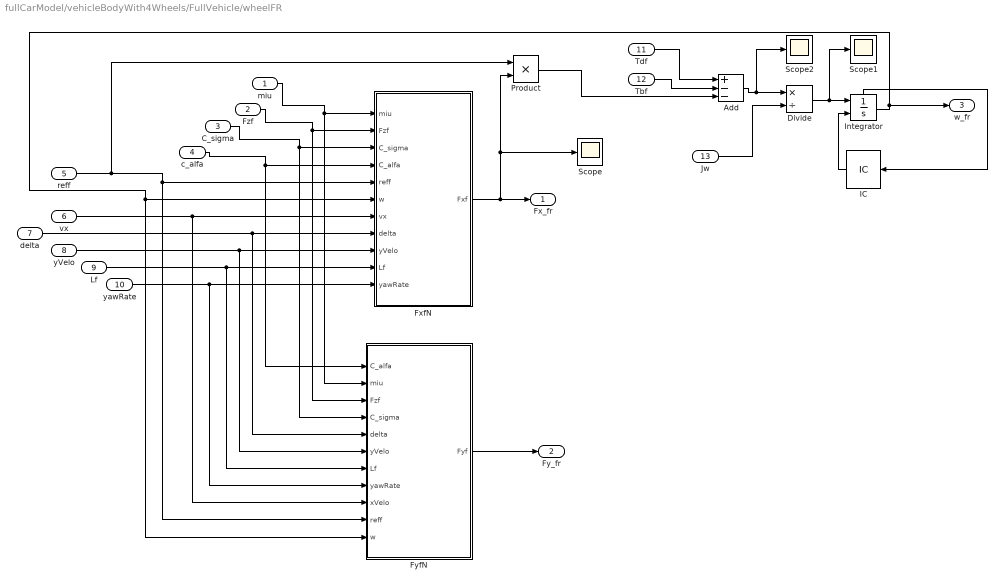
== system fullCarModel/vehicleBodyWith4Wheels/FullVehicle/wheelFR ==
  miu : Inport
  Fzf : Inport  Port=2
  C_sigma : Inport  Port=3
  c_alfa : Inport  Port=4
  reff : Inport  Port=5
  vx : Inport  Port=6
  delta : Inport  Port=7
  yVelo : Inport  Port=8
  Lf : Inport  Port=9
  yawRate : Inport  Port=10
  Tdf : Inport  Port=11
  Tbf : Inport  Port=12
  Jw : Inport  Port=13
  Add : Sum  Inputs=+--
  Divide : Product  Inputs=*/
  FxfN : Subsystem
  FyfN : Subsystem
  IC : InitialCondition  Value=55.55
  Integrator : Integrator  InitialConditionSource=external  ShowStatePort=on
  Product : Product  RndMeth=Zero
  Scope : Scope
  Scope1 : Scope
  Scope2 : Scope
  Fx_fr : Outport
  Fy_fr : Outport  Port=2
  w_fr : Outport  Port=3
  wires:
  miu/1 -> FxfN/1(miu), FyfN/2(miu)
  Fzf/1 -> FxfN/2(Fzf), FyfN/3(Fzf)
  C_sigma/1 -> FxfN/3(C_sigma), FyfN/4(C_sigma)
  c_alfa/1 -> FxfN/4(C_alfa), FyfN/1(C_alfa)
  reff/1 -> FxfN/5(reff), FyfN/10(reff), Product/1
  vx/1 -> FxfN/7(vx), FyfN/9(xVelo)
  delta/1 -> FyfN/5(delta), FxfN/8(delta)
  yVelo/1 -> FyfN/6(yVelo), FxfN/9(yVelo)
  Lf/1 -> FyfN/7(Lf), FxfN/10(Lf)
  yawRate/1 -> FyfN/8(yawRate), FxfN/11(yawRate)
  FxfN/1(Fxf) -> Fx_fr/1, Product/2, Scope/1
  FyfN/1(Fyf) -> Fy_fr/1
  Tdf/1 -> Add/1
  Tbf/1 -> Add/2
  Product/1 -> Add/3
  Jw/1 -> Divide/2
  Add/1 -> Divide/1, Scope2/1
  Divide/1 -> Integrator/1, Scope1/1
  Integrator/1 -> FxfN/6(w), FyfN/11(w), w_fr/1
  IC/1 -> Integrator/2
  Integrator/State -> IC/1

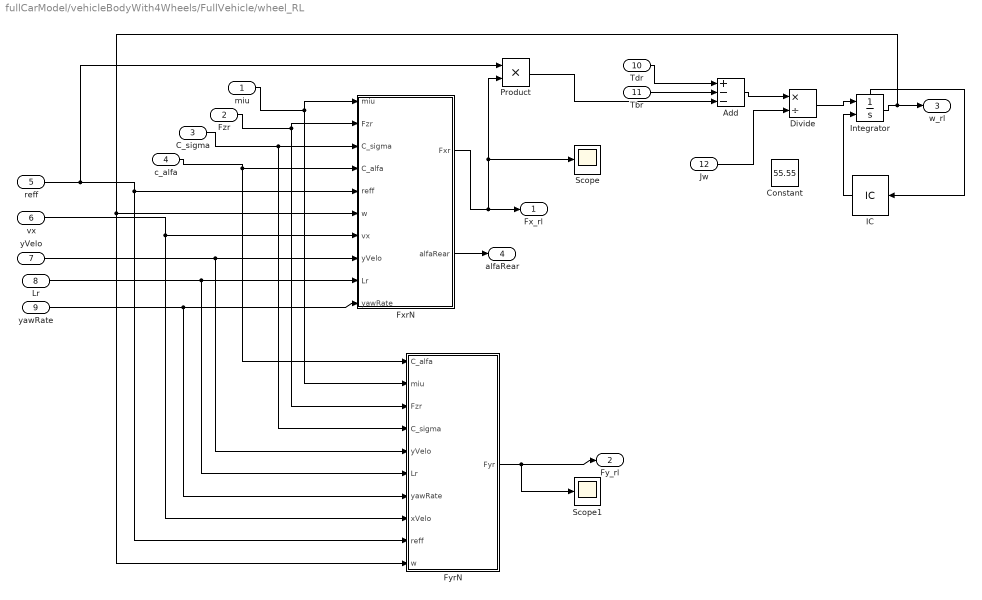
== system fullCarModel/vehicleBodyWith4Wheels/FullVehicle/wheel_RL ==
  miu : Inport
  Fzr : Inport  Port=2
  C_sigma : Inport  Port=3
  c_alfa : Inport  Port=4
  reff : Inport  Port=5
  vx : Inport  Port=6
  yVelo : Inport  Port=7
  Lr : Inport  Port=8
  yawRate : Inport  Port=9
  Tdr : Inport  Port=10
  Tbr : Inport  Port=11
  Jw : Inport  Port=12
  Add : Sum  Inputs=+--
  Constant : Constant  Value=55.55
  Divide : Product  Inputs=*/
  FxrN : Subsystem
  FyrN : Subsystem
  IC : InitialCondition  Value=55.55
  Integrator : Integrator  InitialConditionSource=external  ShowStatePort=on
  Product : Product  RndMeth=Zero
  Scope : Scope
  Scope1 : Scope
  Fx_rl : Outport
  Fy_rl : Outport  Port=2
  w_rl : Outport  Port=3
  alfaRear : Outport  Port=4
  wires:
  miu/1 -> FxrN/1(miu), FyrN/2(miu)
  Fzr/1 -> FxrN/2(Fzr), FyrN/3(Fzr)
  C_sigma/1 -> FxrN/3(C_sigma), FyrN/4(C_sigma)
  c_alfa/1 -> FxrN/4(C_alfa), FyrN/1(C_alfa)
  reff/1 -> FxrN/5(reff), FyrN/9(reff), Product/1
  vx/1 -> FxrN/7(vx), FyrN/8(xVelo)
  yVelo/1 -> FyrN/5(yVelo), FxrN/8(yVelo)
  Lr/1 -> FyrN/6(Lr), FxrN/9(Lr)
  yawRate/1 -> FyrN/7(yawRate), FxrN/10(yawRate)
  Tdr/1 -> Add/1
  Tbr/1 -> Add/2
  Product/1 -> Add/3
  Jw/1 -> Divide/2
  Add/1 -> Divide/1
  Divide/1 -> Integrator/1
  Integrator/1 -> w_rl/1, FxrN/6(w), FyrN/10(w)
  FxrN/1(Fxr) -> Fx_rl/1, Product/2, Scope/1
  FyrN/1(Fyr) -> Scope1/1, Fy_rl/1
  FxrN/2(alfaRear) -> alfaRear/1
  IC/1 -> Integrator/2
  Integrator/State -> IC/1

== system fullCarModel/vehicleBodyWith4Wheels/FullVehicle/wheel_RR ==
  miu : Inport
  Fzr : Inport  Port=2
  C_sigma : Inport  Port=3
  c_alfa : Inport  Port=4
  reff : Inport  Port=5
  vx : Inport  Port=6
  yVelo : Inport  Port=7
  Lr : Inport  Port=8
  yawRate : Inport  Port=9
  Tdr : Inport  Port=10
  Tbr : Inport  Port=11
  Jw : Inport  Port=12
  Add : Sum  Inputs=+--
  Divide : Product  Inputs=*/
  FxrN : Subsystem
  FyrN : Subsystem
  IC : InitialCondition  Value=55.55
  Integrator : Integrator  InitialConditionSource=external  ShowStatePort=on
  Product : Product  RndMeth=Zero
  Scope : Scope
  Fx_rr : Outport
  Fy_rr : Outport  Port=2
  w_rr : Outport  Port=3
  wires:
  miu/1 -> FyrN/2(miu), FxrN/1(miu)
  Fzr/1 -> FyrN/3(Fzr), FxrN/2(Fzr)
  C_sigma/1 -> FyrN/4(C_sigma), FxrN/3(C_sigma)
  c_alfa/1 -> FyrN/1(C_alfa), FxrN/4(C_alfa)
  reff/1 -> FyrN/9(reff), FxrN/5(reff), Product/1
  vx/1 -> FyrN/8(xVelo), FxrN/7(vx)
  yVelo/1 -> FyrN/5(yVelo), FxrN/8(yVelo)
  Lr/1 -> FyrN/6(Lr), FxrN/9(Lr)
  yawRate/1 -> FyrN/7(yawRate), FxrN/10(yawRate)
  Tdr/1 -> Add/1
  Tbr/1 -> Add/2
  Product/1 -> Add/3
  Jw/1 -> Divide/2
  Add/1 -> Divide/1
  Divide/1 -> Integrator/1
  Integrator/1 -> w_rr/1, FyrN/10(w), FxrN/6(w)
  FxrN/1(Fxr) -> Fx_rr/1, Product/2, Scope/1
  FyrN/1(Fyr) -> Fy_rr/1
  IC/1 -> Integrator/2
  Integrator/State -> IC/1

== system fullCarModel/vehicleBodyWith4Wheels/FullVehicle/AirRollWeight/Faero1 ==
  note: Air Drag Faero
  AirDragConst1 : Inport
  FrontalArea1 : Inport  Port=2
  Airdensity : Inport  Port=3
  windVelocity : Inport  Port=4
  Vx : Inport  Port=5
  Add : Sum
  Constant : Constant  Value=0.5
  Math Function : Math  Operator=square  SignedPower=on
  Product : Product  Inputs=5  RndMeth=Zero
  Faero : Outport
  wires:
  FrontalArea1/1 -> Product/2
  Constant/1 -> Product/4
  windVelocity/1 -> Add/1
  Add/1 -> Math Function/1
  Math Function/1 -> Product/5
  Product/1 -> Faero/1
  AirDragConst1/1 -> Product/1
  Airdensity/1 -> Product/3
  Vx/1 -> Add/2

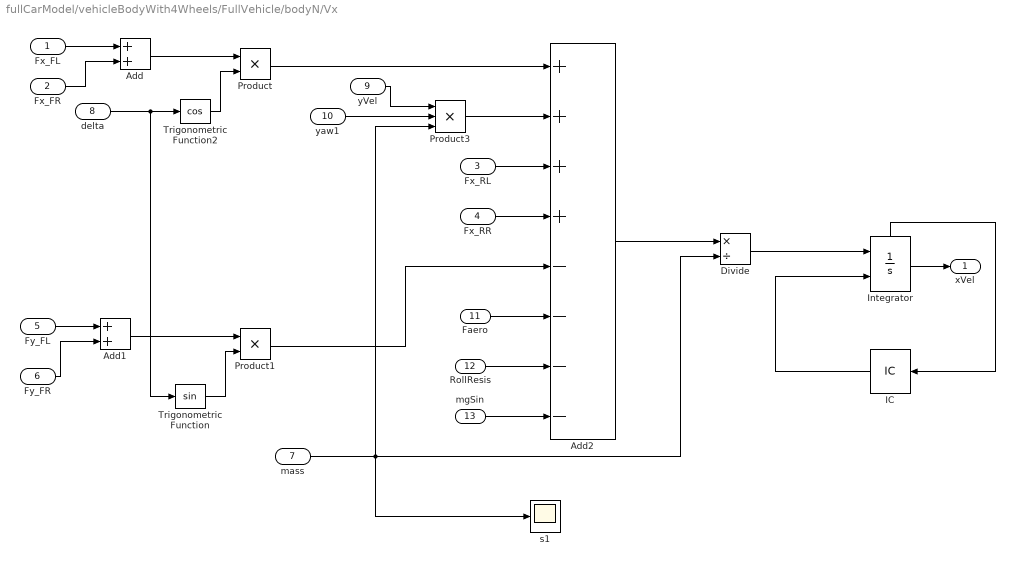
== system fullCarModel/vehicleBodyWith4Wheels/FullVehicle/bodyN/Vx ==
  Fx_FL : Inport
  Fx_FR : Inport  Port=2
  Fx_RL : Inport  Port=3
  Fx_RR : Inport  Port=4
  Fy_FL : Inport  Port=5
  Fy_FR : Inport  Port=6
  mass : Inport  Port=7
  delta : Inport  Port=8
  yVel : Inport  Port=9
  yaw1 : Inport  Port=10
  Faero : Inport  Port=11
  RollResis : Inport  Port=12
  mgSin : Inport  Port=13
  Add : Sum
  Add1 : Sum
  Add2 : Sum  Inputs=++++----
  Divide : Product  Inputs=*/
  IC : InitialCondition  Value=16.666
  Integrator : Integrator  InitialConditionSource=external  InitialCondition=0.0  UpperSaturationLimit=500  LowerSaturationLimit=0.0  ShowStatePort=on
  Product : Product  RndMeth=Zero
  Product1 : Product  RndMeth=Zero
  Product3 : Product  Inputs=3  RndMeth=Zero
  Trigonometric Function : Trigonometry
  Trigonometric Function2 : Trigonometry  Operator=cos
  s1 : Scope
  xVel : Outport
  wires:
  Fx_FL/1 -> Add/1
  Fx_FR/1 -> Add/2
  Add/1 -> Product/1
  Fy_FL/1 -> Add1/1
  Fy_FR/1 -> Add1/2
  Add1/1 -> Product1/1
  Product/1 -> Add2/1
  Add2/1 -> Divide/1
  Divide/1 -> Integrator/1
  delta/1 -> Trigonometric Function2/1, Trigonometric Function/1
  Trigonometric Function2/1 -> Product/2
  Trigonometric Function/1 -> Product1/2
  yVel/1 -> Product3/1
  yaw1/1 -> Product3/2
  Product3/1 -> Add2/2
  Fx_RL/1 -> Add2/3
  Fx_RR/1 -> Add2/4
  Product1/1 -> Add2/5
  Integrator/1 -> xVel/1
  mass/1 -> s1/1, Divide/2, Product3/3
  IC/1 -> Integrator/2
  Integrator/State -> IC/1
  Faero/1 -> Add2/6
  RollResis/1 -> Add2/7
  mgSin/1 -> Add2/8

== system fullCarModel/vehicleBodyWith4Wheels/FullVehicle/bodyN/Vy ==
  Fx_FL : Inport
  Fx_FR : Inport  Port=2
  Fy_RL : Inport  Port=3
  Fy_RR : Inport  Port=4
  Fy_FL : Inport  Port=5
  Fy_FR : Inport  Port=6
  mass : Inport  Port=7
  delta : Inport  Port=8
  xVel : Inport  Port=9
  yaw : Inport  Port=10
  Add : Sum
  Add1 : Sum
  Add2 : Sum  Inputs=+-+++
  Divide : Product  Inputs=*/
  Integrator : Integrator  UpperSaturationLimit=500  LowerSaturationLimit=0  ZeroCross=off
  Product : Product  RndMeth=Zero
  Product1 : Product  RndMeth=Zero
  Product3 : Product  Inputs=3  RndMeth=Zero
  Trigonometric Function : Trigonometry  Operator=cos
  Trigonometric Function2 : Trigonometry
  yVel : Outport
  wires:
  Fx_FL/1 -> Add/1
  Fx_FR/1 -> Add/2
  Add/1 -> Product/1
  Fy_FL/1 -> Add1/1
  Fy_FR/1 -> Add1/2
  Add1/1 -> Product1/1
  mass/1 -> Product3/3, Divide/2
  delta/1 -> Trigonometric Function2/1, Trigonometric Function/1
  Trigonometric Function2/1 -> Product/2
  Trigonometric Function/1 -> Product1/2
  Product3/1 -> Add2/2
  Fy_RL/1 -> Add2/3
  Fy_RR/1 -> Add2/4
  Product1/1 -> Add2/5
  Integrator/1 -> yVel/1
  xVel/1 -> Product3/1
  yaw/1 -> Product3/2
  Product/1 -> Add2/1
  Add2/1 -> Divide/1
  Divide/1 -> Integrator/1

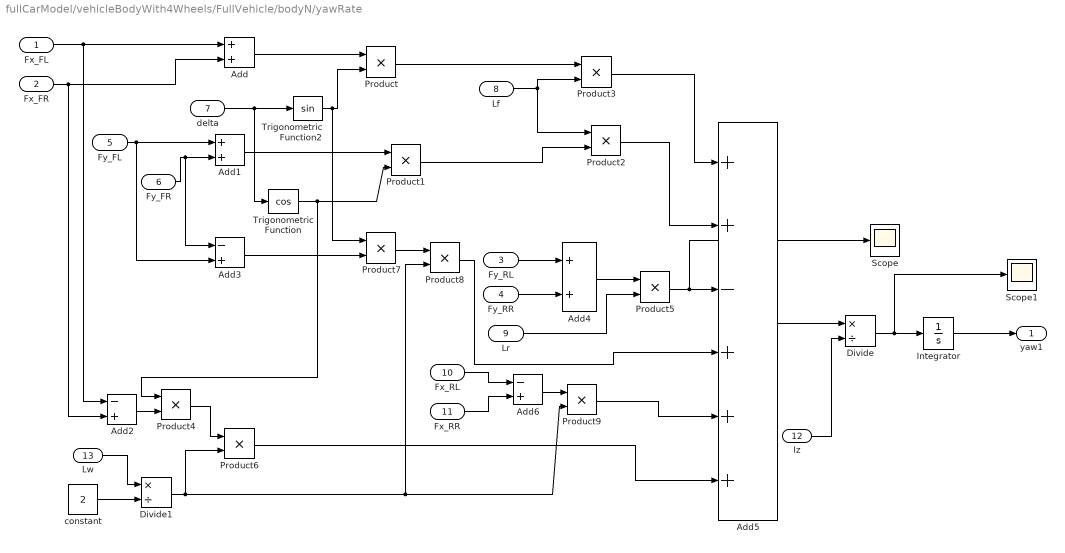
== system fullCarModel/vehicleBodyWith4Wheels/FullVehicle/bodyN/yawRate ==
  Fx_FL : Inport
  Fx_FR : Inport  Port=2
  Fy_RL : Inport  Port=3
  Fy_RR : Inport  Port=4
  Fy_FL : Inport  Port=5
  Fy_FR : Inport  Port=6
  delta : Inport  Port=7
  Lf : Inport  Port=8
  Lr : Inport  Port=9
  Fx_RL : Inport  Port=10
  Fx_RR : Inport  Port=11
  Iz : Inport  Port=12
  Lw : Inport  Port=13
  Add : Sum
  Add1 : Sum
  Add2 : Sum  Inputs=-+
  Add3 : Sum  Inputs=-+
  Add4 : Sum
  Add5 : Sum  Inputs=++-+++
  Add6 : Sum  Inputs=-+
  Divide : Product  Inputs=*/
  Divide1 : Product  Inputs=*/
  Integrator : Integrator  UpperSaturationLimit=500  LowerSaturationLimit=0
  Product{,1..9} (10 alike) : Product  RndMeth=Zero
  Scope : Scope
  Scope1 : Scope
  Trigonometric Function : Trigonometry  Operator=cos
  Trigonometric Function2 : Trigonometry
  constant : Constant  Value=2
  yaw1 : Outport
  wires:
  Fx_FL/1 -> Add/1, Add2/1
  Fx_FR/1 -> Add2/2, Add/2
  Add/1 -> Product/1
  Fy_FL/1 -> Add1/1, Add3/2
  Fy_FR/1 -> Add1/2, Add3/1
  Add1/1 -> Product1/1
  delta/1 -> Trigonometric Function2/1, Trigonometric Function/1
  Trigonometric Function2/1 -> Product/2, Product7/1
  Trigonometric Function/1 -> Product1/2, Product4/1
  Integrator/1 -> yaw1/1
  Fy_RR/1 -> Add4/2
  Fy_RL/1 -> Add4/1
  Product/1 -> Product3/1
  Product1/1 -> Product2/2
  Lf/1 -> Product3/2, Product2/1
  Add4/1 -> Product5/1
  Lr/1 -> Product5/2
  Product3/1 -> Add5/1
  Product2/1 -> Add5/2
  Lw/1 -> Divide1/1
  Add2/1 -> Product4/2
  Product4/1 -> Product6/1
  Divide1/1 -> Product6/2, Product8/2, Product9/2
  Product6/1 -> Add5/6
  Add3/1 -> Product7/2
  Product7/1 -> Product8/1
  Product5/1 -> Add5/3, Scope/1
  Product8/1 -> Add5/4
  Fx_RR/1 -> Add6/2
  Fx_RL/1 -> Add6/1
  Add6/1 -> Product9/1
  Product9/1 -> Add5/5
  Add5/1 -> Divide/1
  Iz/1 -> Divide/2
  Divide/1 -> Integrator/1, Scope1/1
  constant/1 -> Divide1/2

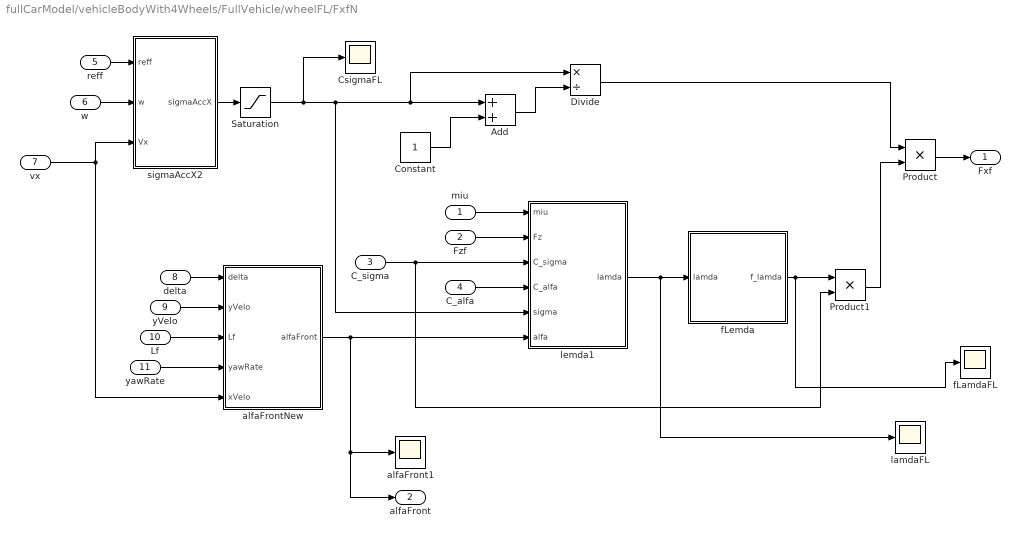
== system fullCarModel/vehicleBodyWith4Wheels/FullVehicle/wheelFL/FxfN ==
  miu : Inport
  Fzf : Inport  Port=2
  C_sigma : Inport  Port=3
  C_alfa : Inport  Port=4
  reff : Inport  Port=5
  w : Inport  Port=6
  vx : Inport  Port=7
  delta : Inport  Port=8
  yVelo : Inport  Port=9
  Lf : Inport  Port=10
  yawRate : Inport  Port=11
  Add : Sum
  Constant : Constant
  CsigmaFL : Scope
  Divide : Product  Inputs=*/
  Product : Product  RndMeth=Zero
  Product1 : Product  RndMeth=Zero
  Saturation : Saturate  UpperLimit=0.15  LowerLimit=0
  alfaFront1 : Scope
  alfaFrontNew : Subsystem
  fLamdaFL : Scope
  fLemda : Subsystem
  lamdaFL : Scope
  lemda1 : Subsystem
  sigmaAccX2 : Subsystem
  Fxf : Outport
  alfaFront : Outport  Port=2
  wires:
  miu/1 -> lemda1/1(miu)
  Fzf/1 -> lemda1/2(Fz)
  C_sigma/1 -> Product1/2, lemda1/3(C_sigma)
  C_alfa/1 -> lemda1/4(C_alfa)
  alfaFrontNew/1(alfaFront) -> lemda1/6(alfa), alfaFront1/1, alfaFront/1
  Constant/1 -> Add/2
  Add/1 -> Divide/2
  Divide/1 -> Product/1
  lemda1/1(lamda) -> fLemda/1(lamda), lamdaFL/1
  fLemda/1(f_lamda) -> Product1/1, fLamdaFL/1
  Product1/1 -> Product/2
  Product/1 -> Fxf/1
  reff/1 -> sigmaAccX2/1(reff)
  w/1 -> sigmaAccX2/2(w)
  vx/1 -> sigmaAccX2/3(Vx), alfaFrontNew/5(xVelo)
  delta/1 -> alfaFrontNew/1(delta)
  yVelo/1 -> alfaFrontNew/2(yVelo)
  Lf/1 -> alfaFrontNew/3(Lf)
  yawRate/1 -> alfaFrontNew/4(yawRate)
  sigmaAccX2/1(sigmaAccX) -> Saturation/1
  Saturation/1 -> CsigmaFL/1, Add/1, Divide/1, lemda1/5(sigma)

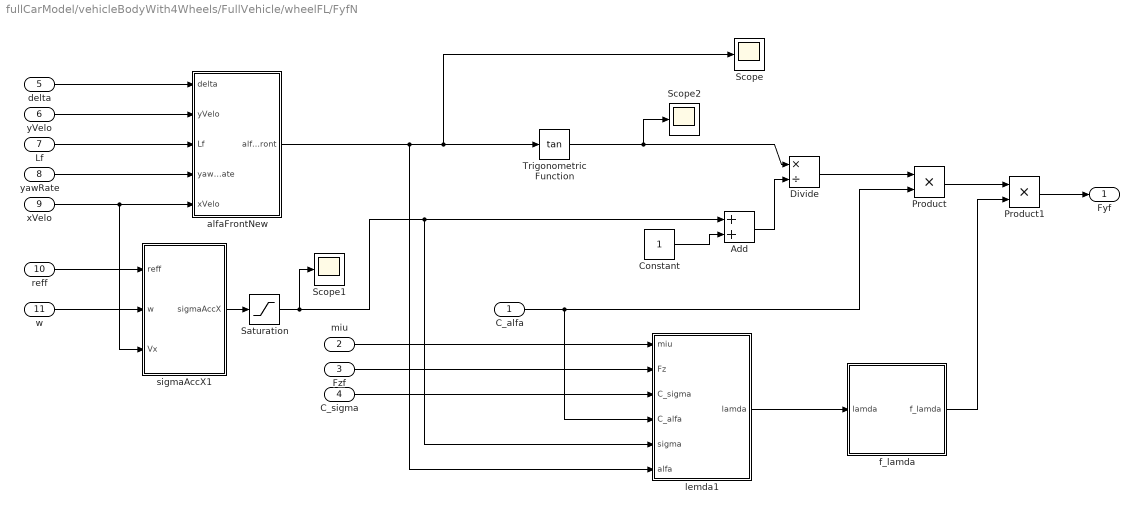
== system fullCarModel/vehicleBodyWith4Wheels/FullVehicle/wheelFL/FyfN ==
  C_alfa : Inport
  miu : Inport  Port=2
  Fzf : Inport  Port=3
  C_sigma : Inport  Port=4
  delta : Inport  Port=5
  yVelo : Inport  Port=6
  Lf : Inport  Port=7
  yawRate : Inport  Port=8
  xVelo : Inport  Port=9
  reff : Inport  Port=10
  w : Inport  Port=11
  Add : Sum
  Constant : Constant
  Divide : Product  Inputs=*/
  Product : Product  RndMeth=Zero
  Product1 : Product  RndMeth=Zero
  Saturation : Saturate  UpperLimit=0.15  LowerLimit=0
  Scope : Scope
  Scope1 : Scope
  Scope2 : Scope
  Trigonometric Function : Trigonometry  Operator=tan
  alfaFrontNew : Subsystem
  f_lamda : Subsystem
  lemda1 : Subsystem
  sigmaAccX1 : Subsystem
  Fyf : Outport
  wires:
  Constant/1 -> Add/2
  alfaFrontNew/1(alfaFront) -> Scope/1, Trigonometric Function/1, lemda1/6(alfa)
  Add/1 -> Divide/2
  Trigonometric Function/1 -> Scope2/1, Divide/1
  C_alfa/1 -> Product/2, lemda1/4(C_alfa)
  Divide/1 -> Product/1
  Product/1 -> Product1/1
  Product1/1 -> Fyf/1
  f_lamda/1(f_lamda) -> Product1/2
  miu/1 -> lemda1/1(miu)
  Fzf/1 -> lemda1/2(Fz)
  C_sigma/1 -> lemda1/3(C_sigma)
  lemda1/1(lamda) -> f_lamda/1(lamda)
  delta/1 -> alfaFrontNew/1(delta)
  yVelo/1 -> alfaFrontNew/2(yVelo)
  Lf/1 -> alfaFrontNew/3(Lf)
  yawRate/1 -> alfaFrontNew/4(yawRate)
  xVelo/1 -> alfaFrontNew/5(xVelo), sigmaAccX1/3(Vx)
  reff/1 -> sigmaAccX1/1(reff)
  w/1 -> sigmaAccX1/2(w)
  sigmaAccX1/1(sigmaAccX) -> Saturation/1
  Saturation/1 -> Scope1/1, Add/1, lemda1/5(sigma)

== system fullCarModel/vehicleBodyWith4Wheels/FullVehicle/wheelFR/FxfN ==
  miu : Inport
  Fzf : Inport  Port=2
  C_sigma : Inport  Port=3
  C_alfa : Inport  Port=4
  reff : Inport  Port=5
  w : Inport  Port=6
  vx : Inport  Port=7
  delta : Inport  Port=8
  yVelo : Inport  Port=9
  Lf : Inport  Port=10
  yawRate : Inport  Port=11
  Add : Sum
  Constant : Constant
  Divide : Product  Inputs=*/
  Product : Product  RndMeth=Zero
  Product1 : Product  RndMeth=Zero
  Saturation : Saturate  UpperLimit=0.15  LowerLimit=0
  Scope : Scope
  alfaFront1 : Scope
  alfaFrontNew : Subsystem
  fLemda : Subsystem
  lamda : Scope
  lemda1 : Subsystem
  sigmaAccX2 : Subsystem
  Fxf : Outport
  wires:
  miu/1 -> lemda1/1(miu)
  Fzf/1 -> lemda1/2(Fz)
  C_sigma/1 -> Product1/2, lemda1/3(C_sigma)
  C_alfa/1 -> lemda1/4(C_alfa)
  alfaFrontNew/1(alfaFront) -> alfaFront1/1, lemda1/6(alfa)
  Constant/1 -> Add/2
  Add/1 -> Divide/2
  Divide/1 -> Product/1, Scope/1
  lemda1/1(lamda) -> lamda/1, fLemda/1(lamda)
  fLemda/1(f_lamda) -> Product1/1
  Product1/1 -> Product/2
  Product/1 -> Fxf/1
  reff/1 -> sigmaAccX2/1(reff)
  w/1 -> sigmaAccX2/2(w)
  vx/1 -> sigmaAccX2/3(Vx), alfaFrontNew/5(xVelo)
  delta/1 -> alfaFrontNew/1(delta)
  yVelo/1 -> alfaFrontNew/2(yVelo)
  Lf/1 -> alfaFrontNew/3(Lf)
  yawRate/1 -> alfaFrontNew/4(yawRate)
  sigmaAccX2/1(sigmaAccX) -> Saturation/1
  Saturation/1 -> Add/1, Divide/1, lemda1/5(sigma)

== system fullCarModel/vehicleBodyWith4Wheels/FullVehicle/wheelFR/FyfN ==
  C_alfa : Inport
  miu : Inport  Port=2
  Fzf : Inport  Port=3
  C_sigma : Inport  Port=4
  delta : Inport  Port=5
  yVelo : Inport  Port=6
  Lf : Inport  Port=7
  yawRate : Inport  Port=8
  xVelo : Inport  Port=9
  reff : Inport  Port=10
  w : Inport  Port=11
  Add : Sum
  Constant : Constant
  Divide : Product  Inputs=*/
  Product : Product  RndMeth=Zero
  Product1 : Product  RndMeth=Zero
  Saturation : Saturate  UpperLimit=0.15  LowerLimit=0
  Trigonometric Function : Trigonometry  Operator=tan
  alfaFrontNew : Subsystem
  f_lamda : Subsystem
  lemda1 : Subsystem
  sigmaAccX2 : Subsystem
  Fyf : Outport
  wires:
  sigmaAccX2/1(sigmaAccX) -> Saturation/1
  Constant/1 -> Add/2
  alfaFrontNew/1(alfaFront) -> Trigonometric Function/1, lemda1/6(alfa)
  Add/1 -> Divide/2
  Trigonometric Function/1 -> Divide/1
  C_alfa/1 -> Product/2, lemda1/4(C_alfa)
  Divide/1 -> Product/1
  Product/1 -> Product1/1
  Product1/1 -> Fyf/1
  f_lamda/1(f_lamda) -> Product1/2
  miu/1 -> lemda1/1(miu)
  Fzf/1 -> lemda1/2(Fz)
  C_sigma/1 -> lemda1/3(C_sigma)
  lemda1/1(lamda) -> f_lamda/1(lamda)
  delta/1 -> alfaFrontNew/1(delta)
  yVelo/1 -> alfaFrontNew/2(yVelo)
  Lf/1 -> alfaFrontNew/3(Lf)
  yawRate/1 -> alfaFrontNew/4(yawRate)
  xVelo/1 -> sigmaAccX2/3(Vx), alfaFrontNew/5(xVelo)
  reff/1 -> sigmaAccX2/1(reff)
  w/1 -> sigmaAccX2/2(w)
  Saturation/1 -> Add/1, lemda1/5(sigma)

== system fullCarModel/vehicleBodyWith4Wheels/FullVehicle/wheel_RL/FxrN ==
  miu : Inport
  Fzr : Inport  Port=2
  C_sigma : Inport  Port=3
  C_alfa : Inport  Port=4
  reff : Inport  Port=5
  w : Inport  Port=6
  vx : Inport  Port=7
  yVelo : Inport  Port=8
  Lr : Inport  Port=9
  yawRate : Inport  Port=10
  Add : Sum
  Constant : Constant
  Divide : Product  Inputs=*/
  Product : Product  RndMeth=Zero
  Product1 : Product  RndMeth=Zero
  Saturation : Saturate  UpperLimit=0.15  LowerLimit=0
  Scope1 : Scope
  alfaRearNew : Subsystem
  f_lamda : Subsystem
  lemda1 : Subsystem
  sigmaAccX2 : Subsystem
  Fxr : Outport
  alfaRear : Outport  Port=2
  wires:
  miu/1 -> lemda1/1(miu)
  Fzr/1 -> lemda1/2(Fz)
  C_sigma/1 -> Product1/2, lemda1/3(C_sigma)
  C_alfa/1 -> lemda1/4(C_alfa)
  alfaRearNew/1(alfaRear) -> lemda1/6(alfa), alfaRear/1
  sigmaAccX2/1(sigmaAccX) -> Saturation/1
  Constant/1 -> Add/2
  Add/1 -> Divide/2
  Divide/1 -> Product/1
  lemda1/1(lamda) -> f_lamda/1(lamda)
  f_lamda/1(f_lamda) -> Product1/1
  Product1/1 -> Product/2
  Product/1 -> Fxr/1
  reff/1 -> sigmaAccX2/1(reff)
  w/1 -> sigmaAccX2/2(w)
  vx/1 -> sigmaAccX2/3(Vx), alfaRearNew/4(xVelo)
  yVelo/1 -> alfaRearNew/1(yVelo)
  Lr/1 -> alfaRearNew/2(Lr)
  yawRate/1 -> alfaRearNew/3(yawRate)
  Saturation/1 -> Scope1/1, Add/1, Divide/1, lemda1/5(sigma)

== system fullCarModel/vehicleBodyWith4Wheels/FullVehicle/wheel_RL/FyrN ==
  C_alfa : Inport
  miu : Inport  Port=2
  Fzr : Inport  Port=3
  C_sigma : Inport  Port=4
  yVelo : Inport  Port=5
  Lr : Inport  Port=6
  yawRate : Inport  Port=7
  xVelo : Inport  Port=8
  reff : Inport  Port=9
  w : Inport  Port=10
  Add : Sum
  Constant : Constant
  Divide : Product  Inputs=*/
  Product : Product  RndMeth=Zero
  Product1 : Product  RndMeth=Zero
  Saturation : Saturate  UpperLimit=0.15  LowerLimit=0
  Scope : Scope
  Scope1 : Scope
  Scope2 : Scope
  Trigonometric Function : Trigonometry  Operator=tan
  alfaRearNew : Subsystem
  f_lamda : Subsystem
  lemda1 : Subsystem
  sigmaAccX2 : Subsystem
  Fyr : Outport
  wires:
  sigmaAccX2/1(sigmaAccX) -> Saturation/1
  Constant/1 -> Add/2
  alfaRearNew/1(alfaRear) -> Trigonometric Function/1, lemda1/6(alfa), Scope/1
  Add/1 -> Divide/2
  Trigonometric Function/1 -> Scope2/1, Divide/1
  C_alfa/1 -> Product/2, lemda1/4(C_alfa)
  Divide/1 -> Product/1
  Product/1 -> Product1/1
  Product1/1 -> Fyr/1
  f_lamda/1(f_lamda) -> Product1/2
  miu/1 -> lemda1/1(miu)
  Fzr/1 -> lemda1/2(Fz)
  C_sigma/1 -> lemda1/3(C_sigma)
  lemda1/1(lamda) -> f_lamda/1(lamda)
  Lr/1 -> alfaRearNew/2(Lr)
  yawRate/1 -> alfaRearNew/3(yawRate)
  xVelo/1 -> sigmaAccX2/3(Vx), alfaRearNew/4(xVelo)
  reff/1 -> sigmaAccX2/1(reff)
  w/1 -> sigmaAccX2/2(w)
  yVelo/1 -> alfaRearNew/1(yVelo)
  Saturation/1 -> Scope1/1, Add/1, lemda1/5(sigma)

== system fullCarModel/vehicleBodyWith4Wheels/FullVehicle/wheel_RR/FxrN ==
  miu : Inport
  Fzr : Inport  Port=2
  C_sigma : Inport  Port=3
  C_alfa : Inport  Port=4
  reff : Inport  Port=5
  w : Inport  Port=6
  vx : Inport  Port=7
  yVelo : Inport  Port=8
  Lr : Inport  Port=9
  yawRate : Inport  Port=10
  Add : Sum
  Constant : Constant
  Divide : Product  Inputs=*/
  Product : Product  RndMeth=Zero
  Product1 : Product  RndMeth=Zero
  Saturation : Saturate  UpperLimit=0.15  LowerLimit=0
  alfaRearNew : Subsystem
  f_lamda : Subsystem
  lemda1 : Subsystem
  sigmaAccX2 : Subsystem
  Fxr : Outport
  wires:
  miu/1 -> lemda1/1(miu)
  Fzr/1 -> lemda1/2(Fz)
  C_sigma/1 -> Product1/2, lemda1/3(C_sigma)
  C_alfa/1 -> lemda1/4(C_alfa)
  alfaRearNew/1(alfaRear) -> lemda1/6(alfa)
  sigmaAccX2/1(sigmaAccX) -> Saturation/1
  Constant/1 -> Add/2
  Add/1 -> Divide/2
  Divide/1 -> Product/1
  lemda1/1(lamda) -> f_lamda/1(lamda)
  f_lamda/1(f_lamda) -> Product1/1
  Product1/1 -> Product/2
  Product/1 -> Fxr/1
  reff/1 -> sigmaAccX2/1(reff)
  w/1 -> sigmaAccX2/2(w)
  vx/1 -> sigmaAccX2/3(Vx), alfaRearNew/4(xVelo)
  yVelo/1 -> alfaRearNew/1(yVelo)
  Lr/1 -> alfaRearNew/2(Lr)
  yawRate/1 -> alfaRearNew/3(yawRate)
  Saturation/1 -> Add/1, Divide/1, lemda1/5(sigma)

== system fullCarModel/vehicleBodyWith4Wheels/FullVehicle/wheel_RR/FyrN ==
  C_alfa : Inport
  miu : Inport  Port=2
  Fzr : Inport  Port=3
  C_sigma : Inport  Port=4
  yVelo : Inport  Port=5
  Lr : Inport  Port=6
  yawRate : Inport  Port=7
  xVelo : Inport  Port=8
  reff : Inport  Port=9
  w : Inport  Port=10
  Add : Sum
  Constant : Constant
  Divide : Product  Inputs=*/
  Product : Product  RndMeth=Zero
  Product1 : Product  RndMeth=Zero
  Saturation : Saturate  UpperLimit=0.15  LowerLimit=0
  Trigonometric Function : Trigonometry  Operator=tan
  alfaRearNew : Subsystem
  f_lamda : Subsystem
  lemda1 : Subsystem
  sigmaAccX2 : Subsystem
  Fyr : Outport
  wires:
  sigmaAccX2/1(sigmaAccX) -> Saturation/1
  Constant/1 -> Add/2
  alfaRearNew/1(alfaRear) -> lemda1/6(alfa), Trigonometric Function/1
  Add/1 -> Divide/2
  Trigonometric Function/1 -> Divide/1
  C_alfa/1 -> Product/2, lemda1/4(C_alfa)
  Divide/1 -> Product/1
  Product/1 -> Product1/1
  Product1/1 -> Fyr/1
  f_lamda/1(f_lamda) -> Product1/2
  miu/1 -> lemda1/1(miu)
  Fzr/1 -> lemda1/2(Fz)
  C_sigma/1 -> lemda1/3(C_sigma)
  lemda1/1(lamda) -> f_lamda/1(lamda)
  Lr/1 -> alfaRearNew/2(Lr)
  yawRate/1 -> alfaRearNew/3(yawRate)
  xVelo/1 -> sigmaAccX2/3(Vx), alfaRearNew/4(xVelo)
  reff/1 -> sigmaAccX2/1(reff)
  w/1 -> sigmaAccX2/2(w)
  yVelo/1 -> alfaRearNew/1(yVelo)
  Saturation/1 -> Add/1, lemda1/5(sigma)

== system fullCarModel/vehicleBodyWith4Wheels/FullVehicle/wheelFL/FxfN/alfaFrontNew ==
  delta : Inport
  yVelo : Inport  Port=2
  Lf : Inport  Port=3
  yawRate : Inport  Port=4
  xVelo : Inport  Port=5
  Add : Sum  Inputs=+-
  Add1 : Sum
  Divide : Product  Inputs=*/
  Product : Product  RndMeth=Zero
  alfaFront : Outport
  wires:
  Lf/1 -> Product/1
  yawRate/1 -> Product/2
  Product/1 -> Add1/2
  yVelo/1 -> Add1/1
  Add1/1 -> Divide/1
  Divide/1 -> Add/2
  delta/1 -> Add/1
  Add/1 -> alfaFront/1
  xVelo/1 -> Divide/2

== system fullCarModel/vehicleBodyWith4Wheels/FullVehicle/wheelFL/FxfN/fLemda ==
  lamda : Inport
  Add : Sum  Inputs=+-
  Constant : Constant  Value=2
  Constant1 : Constant
  If : If  IfExpression=u1< 1  ZeroCross=off
  If Action Subsystem : Subsystem  TreatAsAtomicUnit=on
  If Action Subsystem1 : Subsystem  TreatAsAtomicUnit=on
  Merge : Merge
  Product : Product  RndMeth=Zero
  f_lamda : Outport
  wires:
  lamda/1 -> If/1, Add/2, Product/2
  If/1 -> If Action Subsystem1/Action
  If/2 -> If Action Subsystem/Action
  Constant/1 -> Add/1
  Add/1 -> Product/1
  Product/1 -> If Action Subsystem1/1(In1)
  Constant1/1 -> If Action Subsystem/1(In1)
  If Action Subsystem1/1(Out1) -> Merge/1
  If Action Subsystem/1(Out1) -> Merge/2
  Merge/1 -> f_lamda/1

== system fullCarModel/vehicleBodyWith4Wheels/FullVehicle/wheelFL/FxfN/lemda1 ==
  miu : Inport
  Fz : Inport  Port=2
  C_sigma : Inport  Port=3
  C_alfa : Inport  Port=4
  sigma : Inport  Port=5
  alfa : Inport  Port=6
  Add : Sum
  Add1 : Sum
  Constant : Constant  Value=2
  Constant1 : Constant
  Divide : Product  Inputs=*/
  Math Function : Math  Operator=square  SignedPower=on
  Math Function1 : Math  Operator=square  SignedPower=on
  Product{,1..4} (5 alike) : Product  RndMeth=Zero
  Sqrt : Sqrt
  Trigonometric Function : Trigonometry  Operator=tan
  lamda : Outport
  wires:
  C_alfa/1 -> Product1/1
  alfa/1 -> Trigonometric Function/1
  Trigonometric Function/1 -> Product1/2
  Product/1 -> Math Function/1
  Product1/1 -> Math Function1/1
  Math Function/1 -> Add/1
  Math Function1/1 -> Add/2
  Add/1 -> Sqrt/1
  Sqrt/1 -> Product2/1
  Constant/1 -> Product2/2
  C_sigma/1 -> Product/2
  sigma/1 -> Product/1, Add1/1
  miu/1 -> Product3/1
  Fz/1 -> Product3/2
  Constant1/1 -> Add1/2
  Product3/1 -> Product4/1
  Add1/1 -> Product4/2
  Product4/1 -> Divide/1
  Product2/1 -> Divide/2
  Divide/1 -> lamda/1

== system fullCarModel/vehicleBodyWith4Wheels/FullVehicle/wheelFL/FxfN/sigmaAccX2 ==
  reff : Inport
  w : Inport  Port=2
  Vx : Inport  Port=3
  Add : Sum  Inputs=+-
  Constant : Constant  Value=0.000000001
  Divide : Product  Inputs=*/
  If Action Subsystem2 : Subsystem  TreatAsAtomicUnit=on
  If Action Subsystem3 : Subsystem  TreatAsAtomicUnit=on
  If1 : If
  Merge1 : Merge
  Product : Product  RndMeth=Zero
  Scope : Scope
  Scope1 : Scope
  sigmaAccX : Outport
  wires:
  reff/1 -> Product/1
  Product/1 -> Add/1, Divide/2
  Add/1 -> Divide/1
  w/1 -> Scope1/1, Product/2
  Vx/1 -> Add/2
  Divide/1 -> Scope/1, If Action Subsystem2/1(In1), If1/1
  If1/1 -> If Action Subsystem2/Action
  If1/2 -> If Action Subsystem3/Action
  If Action Subsystem2/1(Out1) -> Merge1/1
  If Action Subsystem3/1(Out1) -> Merge1/2
  Constant/1 -> If Action Subsystem3/1(In1)
  Merge1/1 -> sigmaAccX/1

== system fullCarModel/vehicleBodyWith4Wheels/FullVehicle/wheelFL/FyfN/alfaFrontNew ==
  delta : Inport
  yVelo : Inport  Port=2
  Lf : Inport  Port=3
  yawRate : Inport  Port=4
  xVelo : Inport  Port=5
  Add : Sum  Inputs=+-
  Add1 : Sum
  Divide : Product  Inputs=*/
  Product : Product  RndMeth=Zero
  alfaFront : Outport
  wires:
  Lf/1 -> Product/1
  yawRate/1 -> Product/2
  Product/1 -> Add1/2
  yVelo/1 -> Add1/1
  Add1/1 -> Divide/1
  Divide/1 -> Add/2
  delta/1 -> Add/1
  Add/1 -> alfaFront/1
  xVelo/1 -> Divide/2

== system fullCarModel/vehicleBodyWith4Wheels/FullVehicle/wheelFL/FyfN/f_lamda ==
  lamda : Inport
  Add : Sum  Inputs=+-
  Constant : Constant  Value=2
  Constant1 : Constant
  If : If  IfExpression=u1< 1  ZeroCross=off
  If Action Subsystem : Subsystem  TreatAsAtomicUnit=on
  If Action Subsystem1 : Subsystem  TreatAsAtomicUnit=on
  Merge : Merge
  Product : Product  RndMeth=Zero
  f_lamda : Outport
  wires:
  lamda/1 -> If/1, Add/2, Product/2
  If/1 -> If Action Subsystem1/Action
  If/2 -> If Action Subsystem/Action
  Constant/1 -> Add/1
  Add/1 -> Product/1
  Product/1 -> If Action Subsystem1/1(In1)
  Constant1/1 -> If Action Subsystem/1(In1)
  If Action Subsystem1/1(Out1) -> Merge/1
  If Action Subsystem/1(Out1) -> Merge/2
  Merge/1 -> f_lamda/1

== system fullCarModel/vehicleBodyWith4Wheels/FullVehicle/wheelFL/FyfN/lemda1 ==
  miu : Inport
  Fz : Inport  Port=2
  C_sigma : Inport  Port=3
  C_alfa : Inport  Port=4
  sigma : Inport  Port=5
  alfa : Inport  Port=6
  Add : Sum
  Add1 : Sum
  Constant : Constant  Value=2
  Constant1 : Constant
  Divide : Product  Inputs=*/
  Math Function : Math  Operator=square  SignedPower=on
  Math Function1 : Math  Operator=square  SignedPower=on
  Product{,1..4} (5 alike) : Product  RndMeth=Zero
  Sqrt : Sqrt
  Trigonometric Function : Trigonometry  Operator=tan
  lamda : Outport
  wires:
  C_alfa/1 -> Product1/1
  alfa/1 -> Trigonometric Function/1
  Trigonometric Function/1 -> Product1/2
  Product/1 -> Math Function/1
  Product1/1 -> Math Function1/1
  Math Function/1 -> Add/1
  Math Function1/1 -> Add/2
  Add/1 -> Sqrt/1
  Sqrt/1 -> Product2/1
  Constant/1 -> Product2/2
  C_sigma/1 -> Product/2
  sigma/1 -> Product/1, Add1/1
  miu/1 -> Product3/1
  Fz/1 -> Product3/2
  Constant1/1 -> Add1/2
  Product3/1 -> Product4/1
  Add1/1 -> Product4/2
  Product4/1 -> Divide/1
  Product2/1 -> Divide/2
  Divide/1 -> lamda/1

== system fullCarModel/vehicleBodyWith4Wheels/FullVehicle/wheelFL/FyfN/sigmaAccX1 ==
  reff : Inport
  w : Inport  Port=2
  Vx : Inport  Port=3
  Add : Sum  Inputs=+-
  Constant : Constant  Value=0
  Divide : Product  Inputs=*/
  If Action Subsystem2 : Subsystem  TreatAsAtomicUnit=on
  If Action Subsystem3 : Subsystem  TreatAsAtomicUnit=on
  If1 : If
  Merge1 : Merge
  Product : Product  RndMeth=Zero
  sigmaAccX : Outport
  wires:
  reff/1 -> Product/1
  Product/1 -> Add/1, Divide/2
  Add/1 -> Divide/1
  w/1 -> Product/2
  Vx/1 -> Add/2
  Divide/1 -> If Action Subsystem2/1(In1), If1/1
  If1/1 -> If Action Subsystem2/Action
  If1/2 -> If Action Subsystem3/Action
  If Action Subsystem2/1(Out1) -> Merge1/1
  If Action Subsystem3/1(Out1) -> Merge1/2
  Constant/1 -> If Action Subsystem3/1(In1)
  Merge1/1 -> sigmaAccX/1
